simulink model "Copter_Plane_V10_sim"  (R2021a)
settings: Solver=ode1  StartTime=0.0  StopTime=10  FixedStep=dt  RelTol=1e-3
undefined symbols (not defined in the file or in its folder): AC_Attitude, AC_PosControl, accel_target, AP_Motors, curr_pos, Curr_sate, curr_vel, Euler, GRAVITY_MSS, gyro, HD, J, m_kg, Newton, pid_vel_xy_input, pos_target, position, Raphson, rho, SINS, SRV_Channel, Vehicle, vel_target, velocity
libraries: sharedutil x4, shared6dofsys x2, simulink x2, sharedtransform x2, aerolibasang x1
(part 1 of 2)
settings Model: PauseTimes=0.95  Creator=a4327481  LastModifiedBy=a4327481
settings SolverCC: AlgebraicLoopSolver=TrustRegion
settings DebuggingCC: SFMachineParentedDataDiag=warning

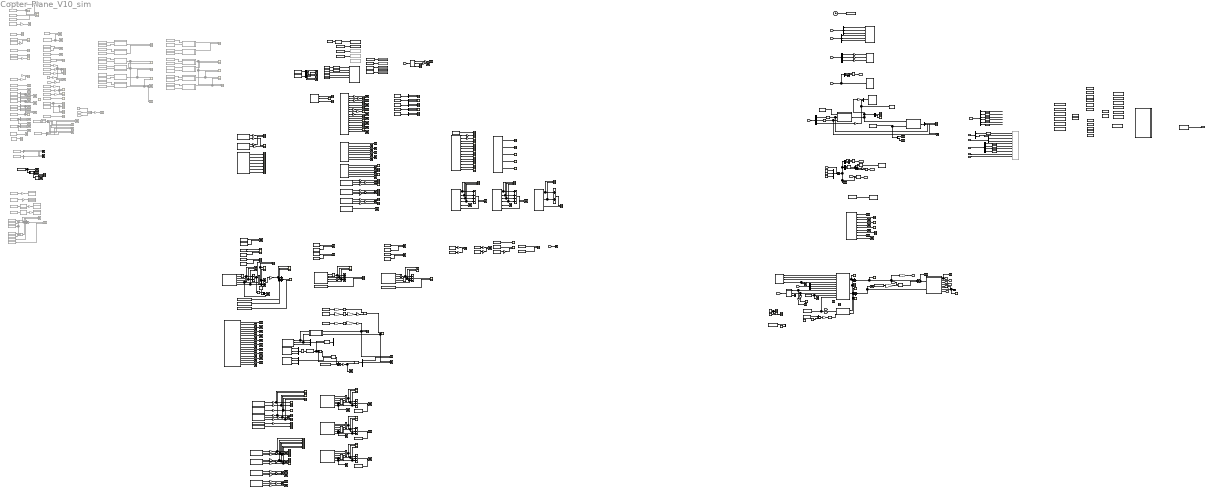
== system Copter_Plane_V10_sim ==
  CTRL_wp : Inport
  PathModeOut : Inport  Port=2  OutDataTypeStr=Bus: BUS_TASK_PATH_OutParam
  TASK_COMMON_OutParam : Inport  Port=3  OutDataTypeStr=Bus: BUS_TASK_COMMON_OutParam
  NAVI2CONTROL : Inport  Port=4  OutDataTypeStr=Bus: BUS_TO_CONTROL
  EAS_Algo : Inport  Port=5  OutDataTypeStr=Bus: BUS_AIRSPEED
  IMU : Inport  Port=6  OutDataTypeStr=Bus: BUS_IMU
  6DOF (Euler Angles) : Subsystem  AncestorBlock=shared6dof/6DOF (Euler Angles)  mask(6DOF EoM (Body Axis)){units=Metric (MKS), mtype=Fixed, rep=Euler Angles, xme_0=position, Vm_0=velocity, eul_0=Euler, pm_0=gyro, mass_0=m_kg, mass_e=0.5, mass_f=2.0, inertia=J, inertia_e=eye(3), inertia_f=2*eye(3), k_quat=1.0, vre_flag=on, abi_flag=off, aMode=0, xme_statename='', Vm_statename='', eul_statename='', quat_statename='', pm_statename='', mass_statename=''}
      mask prompts: units "shared_aeroblks:sharedaeroblk6dofbody:block6DOFEoMBodyAxisParamUnits"; mtype "shared_aeroblks:sharedaeroblk6dofbody:block6DOFEoMBodyAxisParamMasstype"; rep "shared_aeroblks:sharedaeroblk6dofbody:block6DOFEoMBodyAxisParamRepresentation"; xme_0 "shared_aeroblks:sharedaeroblk6dofbody:block6DOFEoMBodyAxisParamInitialpositionininertialaxesXeYeZe"; Vm_0 "shared_aeroblks:sharedaeroblk6dofbody:block6DOFEoMBodyAxisParamInitialvelocityinbodyaxesUvw"; eul_0 "shared_aeroblks:sharedaeroblk6dofbody:block6DOFEoMBodyAxisParamInitialEulerorientationrollpitchyaw"; pm_0 "shared_aeroblks:sharedaeroblk6dofbody:block6DOFEoMBodyAxisParamInitialbodyrotationratespqr"; mass_0 "shared_aeroblks:sharedaeroblk6dofbody:block6DOFEoMBodyAxisParamInitialmass"; mass_e "shared_aeroblks:sharedaeroblk6dofbody:block6DOFEoMBodyAxisParamEmptymass"; mass_f "shared_aeroblks:sharedaeroblk6dofbody:block6DOFEoMBodyAxisParamFullmass"; inertia "shared_aeroblks:sharedaeroblk6dofbody:block6DOFEoMBodyAxisParamInertia"; inertia_e "shared_aeroblks:sharedaeroblk6dofbody:block6DOFEoMBodyAxisParamEmptyinertiamatrix"; inertia_f "shared_aeroblks:sharedaeroblk6dofbody:block6DOFEoMBodyAxisParamFullinertiamatrix"; k_quat "shared_aeroblks:sharedaeroblk6dofbody:block6DOFEoMBodyAxisParamGainforquaternionnormalization"; vre_flag "shared_aeroblks:sharedaeroblk6dofbody:block6DOFEoMBodyAxisParamIncludemassflowrelativevelocity"; abi_flag "shared_aeroblks:sharedaeroblk6dofbody:inertialAccelFlag"; xme_statename "shared_aeroblks:sharedaeroblk6dofbody:block6DOFEoMStateNamePosition"; Vm_statename "shared_aeroblks:sharedaeroblk6dofbody:block6DOFEoMStateNameVelocity"; eul_statename "shared_aeroblks:sharedaeroblk6dofbody:block6DOFEoMStateNameEulerAngles"; quat_statename "shared_aeroblks:sharedaeroblk6dofbody:block6DOFEoMStateNameQuaternions"; pm_statename "shared_aeroblks:sharedaeroblk6dofbody:block6DOFEoMStateNameRotationRates"; mass_statename "shared_aeroblks:sharedaeroblk6dofbody:block6DOFEoMStateNameMass"
      mask help: shared_aeroblks:sharedaeroblk6dofbody:block6DOFEoMBodyAxisDesc
      mask init:
      | if aerosharedtest(gcb)
      |     ports=aerosharedicon('shared6dofbody','icon');
      | else
      |     ports=sharedautoicon('shared6dofbody','icon');
      | end
      mask Help: eval('aerosharedhelp(''sixdof_euler_angles'')');
      mask TypeOptions units: shared_aeroblks:sharedaeroblk6dofbody:block6DOFEoMBodyAxisParamComboMetricMKS | shared_aeroblks:sharedaeroblk6dofbody:block6DOFEoMBodyAxisParamComboEnglishVelocityinfts | shared_aeroblks:sharedaeroblk6dofbody:block6DOFEoMBodyAxisParamComboEnglishVelocityinkts
      mask TypeOptions mtype: shared_aeroblks:sharedaeroblk6dofbody:block6DOFEoMBodyAxisParamComboFixed | shared_aeroblks:sharedaeroblk6dofbody:block6DOFEoMBodyAxisParamComboSimpleVariable | shared_aeroblks:sharedaeroblk6dofbody:block6DOFEoMBodyAxisParamComboCustomVariable
      mask Callback mtype:
      | if aerosharedtest(gcb) && builtin('license','test','aerospace_blockset')
      |     aerosharedicon('shared6dofbody');
      | else
      |     sharedautoicon('shared6dofbody');
      | end
      mask TypeOptions rep: shared_aeroblks:sharedaeroblk6dofbody:block6DOFEoMBodyAxisParamComboEulerAngles | shared_aeroblks:sharedaeroblk6dofbody:block6DOFEoMBodyAxisParamComboQuaternion
      mask Callback rep:
      | if aerosharedtest(gcb) && builtin('license','test','aerospace_blockset')
      |     aerosharedicon('shared6dofbody');
      | else
      |     sharedautoicon('shared6dofbody');
      | end
      mask DialogControl Container4 Prompt: shared_aeroblks:sharedaeroblk6dofbody:block6DOFEoMParamTab
      mask DialogControl units Prompt: Units:
      mask DialogControl mtype Prompt: Mass type:
      mask DialogControl rep Prompt: Representation:
      mask DialogControl xme_0 Prompt: Initial position in inertial axes [Xe,Ye,Ze]:
      mask DialogControl Vm_0 Prompt: Initial velocity in body axes [U,v,w]:
      mask DialogControl eul_0 Prompt: Initial Euler orientation [roll, pitch, yaw]:
      mask DialogControl pm_0 Prompt: Initial body rotation rates [p,q,r]:
      mask DialogControl mass_0 Prompt: Initial mass:
      mask DialogControl mass_e Prompt: Empty mass:
      mask DialogControl mass_f Prompt: Full mass:
      mask DialogControl inertia Prompt: Inertia:
      mask DialogControl inertia_e Prompt: Empty inertia matrix:
      mask DialogControl inertia_f Prompt: Full inertia matrix:
      mask DialogControl k_quat Prompt: Gain for quaternion normalization:
      mask DialogControl vre_flag Prompt: Include mass flow relative velocity
      mask DialogControl abi_flag Prompt: Include inertial acceleration
      mask DialogControl Container6 Prompt: shared_aeroblks:sharedaeroblk6dofbody:block6DOFEoMStateAttributesTab
      mask DialogControl Container7 Prompt: shared_aeroblks:sharedaeroblk6dofbody:block6DOFEoMStateNamesGroup
      mask DialogControl xme_statename Prompt: Position: e.g., {'Xe', 'Ye', 'Ze'}
      mask DialogControl Vm_statename Prompt: Velocity: e.g., {'U', 'v', 'w'}
      mask DialogControl eul_statename Prompt: Euler rotation angles: e.g., {'phi', 'theta', 'psi'}
      mask DialogControl quat_statename Prompt: Quaternion vector: e.g., {'qr', 'qi', 'qj', 'qk'}
      mask DialogControl pm_statename Prompt: Body rotation rates: e.g., {'p', 'q', 'r'}
      mask DialogControl mass_statename Prompt: Mass: e.g., 'mass'
      mask Display:
      | port_label(ports(1).type,ports(1).port,ports(1).txt,'texmode','on');
      | port_label(ports(2).type,ports(2).port,ports(2).txt,'texmode','on');
      | port_label(ports(3).type,ports(3).port,ports(3).txt,'texmode','on');
      | port_label(ports(4).type,ports(4).port,ports(4).txt,'texmode','on');
      | port_label(ports(5).type,ports(5).port,ports(5).txt,'texmode','on');
      | port_label(ports(6).type,ports(6).port,ports(6).txt,'texmode','on');
      | port_label(ports(7).type,ports(7).port,ports(7).txt,'texmode','on');
      | port_label(ports(8).type,ports(8).port,ports(8).txt,'texmode','on');
      | port_label(ports(9).type,ports(9).port,ports(9).txt,'texmode','on');
      | port_label(ports(10).type,ports(10).port,ports(10).txt,'texmode','on');
      | port_label(ports(11).type,ports(11).port,ports(11).txt,'texmode','on');
      | port_label(ports(12).type,ports(12).port,ports(12).txt,'texmode','on');
      | port_label(ports(13).type,ports(13).port,ports(13).txt,'texmode','on');
      | port_label(ports(14).type,ports(14).port,ports(14).txt,'texmode','on');
      | port_label(ports(15).type,ports(15).port,ports(15).txt,'texmode','on');
      | port_label(ports(16).type,ports(16).port,ports(16).txt,'texmode','on');
      | port_label(ports(17).type,ports(17).port,ports(17).txt,'texmode','on');
  AC_Attitude : DataStoreMemory  DataStoreName=AC_Attitude  ReadBeforeWriteMsg=warning  WriteAfterWriteMsg=warning  WriteAfterReadMsg=warning  InitialValue=AC_Attitude  ShowAdditionalParam=off  OutDataTypeStr=Bus: BUS_CTRL_AC_Attitude
  AC_PosControl : DataStoreMemory  DataStoreName=AC_PosControl  ReadBeforeWriteMsg=warning  WriteAfterWriteMsg=warning  WriteAfterReadMsg=warning  InitialValue=AC_PosControl  ShowAdditionalParam=off  OutDataTypeStr=Bus: BUS_CTRL_AC_PosControl
  AC_rate_pitch_pid : DataStoreMemory  DataStoreName=AC_rate_pitch_pid  ReadBeforeWriteMsg=warning  WriteAfterWriteMsg=warning  WriteAfterReadMsg=warning  InitialValue=AC_rate_pitch_pid  ShowAdditionalParam=off  OutDataTypeStr=Bus: BUS_CTRL_PID
  AC_rate_roll_pid : DataStoreMemory  DataStoreName=AC_rate_roll_pid  ReadBeforeWriteMsg=warning  WriteAfterWriteMsg=warning  WriteAfterReadMsg=warning  InitialValue=AC_rate_roll_pid  ShowAdditionalParam=off  OutDataTypeStr=Bus: BUS_CTRL_PID
  AC_rate_yaw_pid : DataStoreMemory  DataStoreName=AC_rate_yaw_pid  ReadBeforeWriteMsg=warning  WriteAfterWriteMsg=warning  WriteAfterReadMsg=warning  InitialValue=AC_rate_yaw_pid  ShowAdditionalParam=off  OutDataTypeStr=Bus: BUS_CTRL_PID
  AP_L1 : DataStoreMemory  DataStoreName=AP_L1  ReadBeforeWriteMsg=warning  WriteAfterWriteMsg=warning  WriteAfterReadMsg=warning  InitialValue=AP_L1  ShowAdditionalParam=off  OutDataTypeStr=Bus: BUS_CTRL_AP_L1
  AP_Motors : DataStoreMemory  DataStoreName=AP_Motors  ReadBeforeWriteMsg=warning  WriteAfterWriteMsg=warning  WriteAfterReadMsg=warning  InitialValue=AP_Motors  VectorParams1D=off  ShowAdditionalParam=off  OutDataTypeStr=Bus: BUS_CTRL_AP_Motors
  AP_TECS : DataStoreMemory  DataStoreName=AP_TECS  ReadBeforeWriteMsg=warning  WriteAfterWriteMsg=warning  WriteAfterReadMsg=warning  InitialValue=AP_TECS  ShowAdditionalParam=off  OutDataTypeStr=Bus: BUS_CTRL_AP_TECS
  AP_rate_pitch : DataStoreMemory  DataStoreName=AP_rate_pitch  ReadBeforeWriteMsg=warning  WriteAfterWriteMsg=warning  WriteAfterReadMsg=warning  InitialValue=AP_rate_pitch  ShowAdditionalParam=off  OutDataTypeStr=Bus: BUS_CTRL_AP_PID_pitch
  AP_rate_roll : DataStoreMemory  DataStoreName=AP_rate_roll  ReadBeforeWriteMsg=warning  WriteAfterWriteMsg=warning  WriteAfterReadMsg=warning  InitialValue=AP_rate_roll  ShowAdditionalParam=off  OutDataTypeStr=Bus: BUS_CTRL_AP_PID_roll
  AP_rate_yaw : DataStoreMemory  DataStoreName=AP_rate_yaw  ReadBeforeWriteMsg=warning  WriteAfterWriteMsg=warning  WriteAfterReadMsg=warning  InitialValue=AP_rate_yaw  ShowAdditionalParam=off  OutDataTypeStr=Bus: BUS_CTRL_AP_PID_yaw
  Add : Sum  Inputs=++++
  Add{1,3,5,7,9,15..16} (7 alike) : Sum
  Add{4,6,10..13} (6 alike) : Sum  Inputs=+++
  Add14 : Sum  Inputs=++++
  Add2 : Sum  Commented=on  Inputs=+++
  Add8 : Sum  Inputs=+-
  Atan1 : Trigonometry  Operator=atan2
  Atan3 : Trigonometry  Operator=atan2
  Atan4 : Trigonometry  Operator=atan2
  Bus Selector : BusSelector  OutputSignals=curVelNED,curLLA
  Bus Selector1 : BusSelector  OutputSignals=pitchd,rolld,yawd,alt
  Bus Selector2 : BusSelector  OutputSignals=gyro_x,gyro_y,gyro_z,accel_x,accel_y,accel_z
  Bus Selector3 : BusSelector  OutputSignals=airspeed_indicate,EAS2TAS_Algo
  Clock : Clock
  Constant : Constant  Value=[40,100]*1e7
  Constant1 : Constant  Value=500/4500*0.95+0.05
  Constant10 : Constant  Value=500/4500*0.95+0.05
  Constant11 : Constant  Value=[40,100]*1e7
  Constant12 : Constant  Value=0
  Constant13 : Constant  Value=0
  Constant14 : Constant  Value=2  OutDataTypeStr=double
  Constant15 : Constant  Value=50  OutDataTypeStr=double
  Constant16 : Constant  OutDataTypeStr=double
  Constant17 : Constant  Value=[1750 1250 1750 1250]  VectorParams1D=off
  Constant2 : Constant  Value=1000  VectorParams1D=off
  Constant27 : Constant  Value=10  OutDataTypeStr=int16
  Constant3 : Constant  Value=[1 1 1 1]'
  Constant30 : Constant  Value=0
  Constant4 : Constant  Value=[1000 1000]
  Constant5 : Constant  Value=rho
  Constant6 : Constant  Value=4  OutDataTypeStr=int16
  Constant7 : Constant  Value=(1/rho)^0.5
  Constant8 : Constant  Value=11  OutDataTypeStr=int16
  Constant9 : Constant  Value=0.4
  Copter_Plane : DataStoreMemory  DataStoreName=Copter_Plane  ReadBeforeWriteMsg=warning  WriteAfterWriteMsg=warning  WriteAfterReadMsg=warning  InitialValue=Copter_Plane  VectorParams1D=off  ShowAdditionalParam=off  OutDataTypeStr=Bus: BUS_CTRL_Copter_Plane
  Curr_sate : DataStoreMemory  DataStoreName=Curr_sate  ReadBeforeWriteMsg=warning  WriteAfterWriteMsg=warning  WriteAfterReadMsg=warning  InitialValue=Curr_sate  VectorParams1D=off  ShowAdditionalParam=off  OutDataTypeStr=Bus: BUS_CTRL_Curr_sate
  Data Store Read : DataStoreRead  DataStoreName=SRV_Channel  IndexOptions=Index vector (dialog)  Indices=1  OutputSizes=1
  Data Store Read1 : DataStoreRead  DataStoreName=SINS  DataStoreElements=SINS.gyro_x#SINS.gyro_y#SINS.gyro_z#SINS.accel_x#SINS.accel_y#SINS.accel_z#SINS.roll#SINS.pitch#SINS.yaw#SINS.curr_vel(:,:)#SINS.curr_loc(:,:)#SINS.curr_alt#SINS.aspeed#SINS.EAS2TAS#SINS.groundspeed_vector(:,:)#SINS.curr_pos(:,:)#SINS.z_accel_meas  IndexOptions=Index vector (dialog)  Indices=1  OutputSizes=1
  Data Store Read10 : DataStoreRead  DataStoreName=AC_PosControl  DataStoreElements=AC_PosControl.vel_target(:,2)  IndexOptions=Index vector (dialog)  Indices=1  OutputSizes=1
  Data Store Read100 : DataStoreRead  DataStoreName=AP_rate_pitch  DataStoreElements=AP_rate_pitch.pid_info_P#AP_rate_pitch.pid_info_I#AP_rate_pitch.pid_info_D#AP_rate_pitch.pid_info_FF#AP_rate_pitch.pid_info_Dmod#AP_rate_pitch.last_out  IndexOptions=Index vector (dialog)  Indices=1  OutputSizes=1
  Data Store Read101 : DataStoreRead  DataStoreName=AP_rate_yaw  DataStoreElements=AP_rate_yaw.pid_info_I#AP_rate_yaw.pid_info_D#AP_rate_yaw.last_out  IndexOptions=Index vector (dialog)  Indices=1  OutputSizes=1
  Data Store Read102 : DataStoreRead  Commented=on  DataStoreName=pos_target  DataStoreElements=pos_target(:,1)  IndexOptions=Index vector (dialog)  Indices=1  OutputSizes=1
  Data Store Read103 : DataStoreRead  Commented=on  DataStoreName=curr_vel  DataStoreElements=curr_vel(:,1)  IndexOptions=Index vector (dialog)  Indices=1  OutputSizes=1
  Data Store Read104 : DataStoreRead  Commented=on  DataStoreName=curr_vel  DataStoreElements=curr_vel(:,2)  IndexOptions=Index vector (dialog)  Indices=1  OutputSizes=1
  Data Store Read105 : DataStoreRead  DataStoreName=AP_L1  DataStoreElements=AP_L1.L1_dist#AP_L1.last_Nu#AP_L1.latAccDem#AP_L1.nav_bearing#AP_L1.bearing_error  IndexOptions=Index vector (dialog)  Indices=1  OutputSizes=1
  Data Store Read106 : DataStoreRead  Commented=on  DataStoreName=thrust_error_angle  IndexOptions=Index vector (dialog)  Indices=1  OutputSizes=1
  Data Store Read107 : DataStoreRead  DataStoreName=AC_PosControl  DataStoreElements=AC_PosControl.accel_desired(:,:)  IndexOptions=Index vector (dialog)  Indices=1  OutputSizes=1
  Data Store Read108 : DataStoreRead  DataStoreName=AC_PosControl  DataStoreElements=AC_PosControl.accel_target(:,:)  IndexOptions=Index vector (dialog)  Indices=1  OutputSizes=1
  Data Store Read109 : DataStoreRead  DataStoreName=SINS  DataStoreElements=SINS.curr_vel(:,:)  IndexOptions=Index vector (dialog)  Indices=1  OutputSizes=1
  Data Store Read11 : DataStoreRead  DataStoreName=AC_PosControl  DataStoreElements=AC_PosControl.pos_target(:,2)  IndexOptions=Index vector (dialog)  Indices=1  OutputSizes=1
  Data Store Read110 : DataStoreRead  Commented=on  DataStoreName=nav_bearing  IndexOptions=Index vector (dialog)  Indices=1  OutputSizes=1
  Data Store Read111 : DataStoreRead  DataStoreName=SRV_Channel  DataStoreElements=SRV_Channel.k_rudder#SRV_Channel.k_aileron#SRV_Channel.k_throttle#SRV_Channel.k_elevator  IndexOptions=Index vector (dialog)  Indices=1  OutputSizes=1
  Data Store Read112 : DataStoreRead  DataStoreName=AC_PosControl  DataStoreElements=AC_PosControl.vel_target(:,:)  IndexOptions=Index vector (dialog)  Indices=1  OutputSizes=1
  Data Store Read113 : DataStoreRead  Commented=on  DataStoreName=mode_L1  IndexOptions=Index vector (dialog)  Indices=1  OutputSizes=1
  Data Store Read114 : DataStoreRead  DataStoreName=AC_PosControl  DataStoreElements=AC_PosControl.accel_target(:,3)  IndexOptions=Index vector (dialog)  Indices=1  OutputSizes=1
  Data Store Read115 : DataStoreRead  Commented=on  DataStoreName=pid_vel_xy_input  DataStoreElements=pid_vel_xy_input(:,1)  IndexOptions=Index vector (dialog)  Indices=1  OutputSizes=1
  Data Store Read116 : DataStoreRead  DataStoreName=SINS  DataStoreElements=SINS.z_accel_meas  IndexOptions=Index vector (dialog)  Indices=1  OutputSizes=1
  Data Store Read117 : DataStoreRead  DataStoreName=SINS  DataStoreElements=SINS.curr_vel(:,3)  IndexOptions=Index vector (dialog)  Indices=1  OutputSizes=1
  Data Store Read118 : DataStoreRead  DataStoreName=AC_PosControl  DataStoreElements=AC_PosControl.vel_desired(:,3)#AC_PosControl.vel_target(:,3)  IndexOptions=Index vector (dialog)  Indices=1  OutputSizes=1
  Data Store Read119 : DataStoreRead  DataStoreName=AC_PosControl  DataStoreElements=AC_PosControl.pos_target(:,3)  IndexOptions=Index vector (dialog)  Indices=1  OutputSizes=1
  Data Store Read12 : DataStoreRead  Commented=on  DataStoreName=pwm_out  IndexOptions=Index vector (dialog)  Indices=1  OutputSizes=1
  Data Store Read120 : DataStoreRead  DataStoreName=SINS  DataStoreElements=SINS.curr_alt  IndexOptions=Index vector (dialog)  Indices=1  OutputSizes=1
  Data Store Read121 : DataStoreRead  Commented=on  DataStoreName=z_accel_meas  IndexOptions=Index vector (dialog)  Indices=1  OutputSizes=1
  Data Store Read122 : DataStoreRead  Commented=on  DataStoreName=latAccDem  IndexOptions=Index vector (dialog)  Indices=1  OutputSizes=1
  Data Store Read123 : DataStoreRead  DataStoreName=AC_PosControl  DataStoreElements=AC_PosControl.vel_target(:,1)  IndexOptions=Index vector (dialog)  Indices=1  OutputSizes=1
  Data Store Read124 : DataStoreRead  DataStoreName=AC_PosControl  DataStoreElements=AC_PosControl.pos_target(:,1)  IndexOptions=Index vector (dialog)  Indices=1  OutputSizes=1
  Data Store Read125 : DataStoreRead  DataStoreName=SINS  DataStoreElements=SINS.curr_pos(:,1)  IndexOptions=Index vector (dialog)  Indices=1  OutputSizes=1
  Data Store Read126 : DataStoreRead  Commented=on  DataStoreName=pwm_out  IndexOptions=Index vector (dialog)  Indices=1  OutputSizes=1
  Data Store Read127 : DataStoreRead  Commented=on  DataStoreName=pos_target  IndexOptions=Index vector (dialog)  Indices=1  OutputSizes=1
  Data Store Read128 : DataStoreRead  Commented=on  DataStoreName=vel_target  IndexOptions=Index vector (dialog)  Indices=1  OutputSizes=1
  Data Store Read129 : DataStoreRead  Commented=on  DataStoreName=vel_desired  IndexOptions=Index vector (dialog)  Indices=1  OutputSizes=1
  Data Store Read13 : DataStoreRead  Commented=on  DataStoreName=thrust_rpyt_out  IndexOptions=Index vector (dialog)  Indices=1  OutputSizes=1
  Data Store Read130 : DataStoreRead  Commented=on  DataStoreName=accel_target  IndexOptions=Index vector (dialog)  Indices=1  OutputSizes=1
  Data Store Read131 : DataStoreRead  Commented=on  DataStoreName=accel_desired  IndexOptions=Index vector (dialog)  Indices=1  OutputSizes=1
  Data Store Read132 : DataStoreRead  DataStoreName=AP_Motors  DataStoreElements=AP_Motors.throttle_hover  IndexOptions=Index vector (dialog)  Indices=1  OutputSizes=1
  Data Store Read133 : DataStoreRead  Commented=on  DataStoreName=EAS_dem  IndexOptions=Index vector (dialog)  Indices=1  OutputSizes=1
  Data Store Read134 : DataStoreRead  Commented=on  DataStoreName=nav_pitch_cd  IndexOptions=Index vector (dialog)  Indices=1  OutputSizes=1
  Data Store Read135 : DataStoreRead  DataStoreName=AP_Motors  DataStoreElements=AP_Motors.throttle_in  IndexOptions=Index vector (dialog)  Indices=1  OutputSizes=1
  Data Store Read136 : DataStoreRead  Commented=on  DataStoreName=nav_roll_cd  IndexOptions=Index vector (dialog)  Indices=1  OutputSizes=1
  Data Store Read137 : DataStoreRead  DataStoreName=AP_Motors  DataStoreElements=AP_Motors.angle_boost  IndexOptions=Index vector (dialog)  Indices=1  OutputSizes=1
  Data Store Read138 : DataStoreRead  DataStoreName=AC_Attitude  DataStoreElements=AC_Attitude.rate_target_ang_vel(:,1)#AC_Attitude.rate_target_ang_vel(:,2)#AC_Attitude.rate_target_ang_vel(:,3)  IndexOptions=Index vector (dialog)  Indices=1  OutputSizes=1
  Data Store Read139 : DataStoreRead  DataStoreName=SINS  DataStoreElements=SINS.curr_pos(:,2)  IndexOptions=Index vector (dialog)  Indices=1  OutputSizes=1
  Data Store Read14 : DataStoreRead  DataStoreName=SRV_Channel  DataStoreElements=SRV_Channel.k_rudder#SRV_Channel.k_aileron#SRV_Channel.k_elevator#SRV_Channel.k_throttle#SRV_Channel.k_flap#SRV_Channel.tail_tilt#SRV_Channel.pwm_tail#SRV_Channel.pwm_out(:,:)  IndexOptions=Index vector (dialog)  Indices=1  OutputSizes=1
  Data Store Read140 : DataStoreRead  DataStoreName=SINS  DataStoreElements=SINS.curr_vel(:,2)  IndexOptions=Index vector (dialog)  Indices=1  OutputSizes=1
  Data Store Read141 : DataStoreRead  DataStoreName=SINS  DataStoreElements=SINS.gyro_x#SINS.gyro_y#SINS.gyro_z  IndexOptions=Index vector (dialog)  Indices=1  OutputSizes=1
  Data Store Read142 : DataStoreRead  DataStoreName=SINS  DataStoreElements=SINS.roll#SINS.pitch#SINS.yaw  IndexOptions=Index vector (dialog)  Indices=1  OutputSizes=1
  Data Store Read143 : DataStoreRead  Commented=on  DataStoreName=roll  IndexOptions=Index vector (dialog)  Indices=1  OutputSizes=1
  Data Store Read144 : DataStoreRead  DataStoreName=SINS  DataStoreElements=SINS.curr_alt  IndexOptions=Index vector (dialog)  Indices=1  OutputSizes=1
  Data Store Read145 : DataStoreRead  DataStoreName=SINS  DataStoreElements=SINS.aspeed  IndexOptions=Index vector (dialog)  Indices=1  OutputSizes=1
  Data Store Read146 : DataStoreRead  DataStoreName=AP_TECS  DataStoreElements=AP_TECS.TAS_dem_adj  IndexOptions=Index vector (dialog)  Indices=1  OutputSizes=1
  Data Store Read147 : DataStoreRead  DataStoreName=SRV_Channel  DataStoreElements=SRV_Channel.k_throttle  IndexOptions=Index vector (dialog)  Indices=1  OutputSizes=1
  Data Store Read148 : DataStoreRead  DataStoreName=AC_Attitude  DataStoreElements=AC_Attitude.attitude_target_ang_vel(:,1)#AC_Attitude.attitude_target_ang_vel(:,2)#AC_Attitude.attitude_target_ang_vel(:,3)  IndexOptions=Index vector (dialog)  Indices=1  OutputSizes=1
  Data Store Read149 : DataStoreRead  DataStoreName=AC_Attitude  DataStoreElements=AC_Attitude.attitude_target_quat(:,:)  IndexOptions=Index vector (dialog)  Indices=1  OutputSizes=1
  Data Store Read15 : DataStoreRead  DataStoreName=AP_Motors  DataStoreElements=AP_Motors.yaw_in  IndexOptions=Index vector (dialog)  Indices=1  OutputSizes=1
  Data Store Read150 : DataStoreRead  Commented=on  DataStoreName=pid_info_I_pitch  IndexOptions=Index vector (dialog)  Indices=1  OutputSizes=1
  Data Store Read151 : DataStoreRead  Commented=on  DataStoreName=last_out_pitch  IndexOptions=Index vector (dialog)  Indices=1  OutputSizes=1
  Data Store Read152 : DataStoreRead  DataStoreName=AC_Attitude  DataStoreElements=AC_Attitude.attitude_target_euler_rate(:,1)#AC_Attitude.attitude_target_euler_rate(:,2)#AC_Attitude.attitude_target_euler_rate(:,3)  IndexOptions=Index vector (dialog)  Indices=1  OutputSizes=1
  Data Store Read153 : DataStoreRead  Commented=on  DataStoreName=pid_vel_xy_input  DataStoreElements=pid_vel_xy_input(:,2)  IndexOptions=Index vector (dialog)  Indices=1  OutputSizes=1
  Data Store Read154 : DataStoreRead  DataStoreName=SlewLimiter  DataStoreElements=SlewLimiter.pos_event_stored#SlewLimiter.neg_event_stored#SlewLimiter.pos_event_index#SlewLimiter.neg_event_index#SlewLimiter.pos_event_ms(:,:)#SlewLimiter.neg_event_ms(:,:)#SlewLimiter.max_pos_slew_rate#SlewLimiter.max_neg_slew_rate#SlewLimiter.modifier_slew_rate#SlewLimiter.output_slew_rate#SlewLimiter.last_sample#SlewLimiter.slew_filter#SlewLimiter.N_EVENTS#SlewLimiter.max_pos_slew_event_ms#SlewLimiter.max_neg_slew_event_ms#SlewLimiter.MODIFIER_GAIN#SlewLimiter.WINDOW_MS#SlewLimiter.DERIVATIVE_CUTOFF_FREQ#SlewLimiter.slew_rate_max#SlewLimiter.slew_rate_tau  IndexOptions=Index vector (dialog)  Indices=1  OutputSizes=1
  Data Store Read158 : DataStoreRead  Commented=on  DataStoreName=attitude_target_quat  IndexOptions=Index vector (dialog)  Indices=1  OutputSizes=1
  Data Store Read159 : DataStoreRead  Commented=on  DataStoreName=rate_pitch_pid  DataStoreElements=rate_pitch_pid.kp  IndexOptions=Index vector (dialog)  Indices=1  OutputSizes=1
  Data Store Read16 : DataStoreRead  DataStoreName=SINS  DataStoreElements=SINS.aspeed  IndexOptions=Index vector (dialog)  Indices=1  OutputSizes=1
  Data Store Read160 : DataStoreRead  Commented=on  DataStoreName=rate_pitch_pid  DataStoreElements=rate_pitch_pid.error  IndexOptions=Index vector (dialog)  Indices=1  OutputSizes=1
  Data Store Read163 : DataStoreRead  Commented=on  DataStoreName=rate_pitch_pid  DataStoreElements=rate_pitch_pid.kd  IndexOptions=Index vector (dialog)  Indices=1  OutputSizes=1
  Data Store Read164 : DataStoreRead  Commented=on  DataStoreName=rate_pitch_pid  DataStoreElements=rate_pitch_pid.derivative  IndexOptions=Index vector (dialog)  Indices=1  OutputSizes=1
  Data Store Read165 : DataStoreRead  Commented=on  DataStoreName=rate_pitch_pid  DataStoreElements=rate_pitch_pid.integrator  IndexOptions=Index vector (dialog)  Indices=1  OutputSizes=1
  Data Store Read166 : DataStoreRead  DataStoreName=AC_PosControl  DataStoreElements=AC_PosControl.roll_target#AC_PosControl.pitch_target  IndexOptions=Index vector (dialog)  Indices=1  OutputSizes=1
  Data Store Read167 : DataStoreRead  DataStoreName=AC_Attitude  DataStoreElements=AC_Attitude.attitude_target_euler_angle(:,3)  IndexOptions=Index vector (dialog)  Indices=1  OutputSizes=1
  Data Store Read168 : DataStoreRead  Commented=on  DataStoreName=rate_pitch_pid  DataStoreElements=rate_pitch_pid.Dmod  IndexOptions=Index vector (dialog)  Indices=1  OutputSizes=1
  Data Store Read169 : DataStoreRead  Commented=on  DataStoreName=pitch_in  IndexOptions=Index vector (dialog)  Indices=1  OutputSizes=1
  Data Store Read17 : DataStoreRead  DataStoreName=SRV_Channel  DataStoreElements=SRV_Channel.pwm_out(:,1:2)  IndexOptions=Index vector (dialog)  Indices=1  OutputSizes=1
  Data Store Read171 : DataStoreRead  DataStoreName=SINS  DataStoreElements=SINS.accel_x#SINS.accel_y#SINS.accel_z  IndexOptions=Index vector (dialog)  Indices=1  OutputSizes=1
  Data Store Read172 : DataStoreRead  DataStoreName=AC_PosControl  DataStoreElements=AC_PosControl.accel_target(:,1)#AC_PosControl.accel_target(:,2)#AC_PosControl.accel_target(:,3)  IndexOptions=Index vector (dialog)  Indices=1  OutputSizes=1
  Data Store Read174 : DataStoreRead  DataStoreName=SINS  DataStoreElements=SINS.roll#SINS.pitch#SINS.yaw  IndexOptions=Index vector (dialog)  Indices=1  OutputSizes=1
  Data Store Read18 : DataStoreRead  DataStoreName=plane_mode  IndexOptions=Index vector (dialog)  Indices=1  OutputSizes=1
  Data Store Read19 : DataStoreRead  DataStoreName=AP_Motors  DataStoreElements=AP_Motors.thrust_rpyt_out(:,:)#AP_Motors.throttle_filter#AP_Motors.roll_in#AP_Motors.pitch_in#AP_Motors.yaw_in#AP_Motors.throttle_in  IndexOptions=Index vector (dialog)  Indices=1  OutputSizes=1
  Data Store Read2 : DataStoreRead  Commented=on  DataStoreName=pid_info_P_pitch  IndexOptions=Index vector (dialog)  Indices=1  OutputSizes=1
  Data Store Read20 : DataStoreRead  Commented=on  DataStoreName=pitch  IndexOptions=Index vector (dialog)  Indices=1  OutputSizes=1
  Data Store Read21 : DataStoreRead  DataStoreName=Test_w  DataStoreElements=Test_w.roll_in#Test_w.pitch_in#Test_w.yaw_in#Test_w.throttle_in#Test_w.k_rudder#Test_w.k_elevator#Test_w.k_throttle#Test_w.k_aileron#Test_w.k_flap#Test_w.out  IndexOptions=Index vector (dialog)  Indices=1  OutputSizes=1
  Data Store Read22 : DataStoreRead  DataStoreName=Plane  DataStoreElements=Plane.nav_roll_cd#Plane.nav_pitch_cd  IndexOptions=Index vector (dialog)  Indices=1  OutputSizes=1
  Data Store Read23 : DataStoreRead  DataStoreName=SINS  DataStoreElements=SINS.roll#SINS.pitch#SINS.yaw  IndexOptions=Index vector (dialog)  Indices=1  OutputSizes=1
  Data Store Read24 : DataStoreRead  DataStoreName=AP_rate_pitch  DataStoreElements=AP_rate_pitch.pid_info_target#AP_rate_pitch.pid_info_actual#AP_rate_pitch.pid_info_error#AP_rate_pitch.pid_info_P#AP_rate_pitch.pid_info_I#AP_rate_pitch.pid_info_FF#AP_rate_pitch.pid_info_D  IndexOptions=Index vector (dialog)  Indices=1  OutputSizes=1
  Data Store Read25 : DataStoreRead  DataStoreName=PathModeOut_sl  DataStoreElements=PathModeOut_sl.flightControlMode  IndexOptions=Index vector (dialog)  Indices=1  OutputSizes=1
  Data Store Read26 : DataStoreRead  DataStoreName=Copter_Plane  DataStoreElements=Copter_Plane.roll_target_pilot#Copter_Plane.pitch_target_pilot#Copter_Plane.climb_rate_cms  IndexOptions=Index vector (dialog)  Indices=1  OutputSizes=1
  Data Store Read27 : DataStoreRead  DataStoreName=AC_PosControl  DataStoreElements=AC_PosControl.accel_target(:,1)  IndexOptions=Index vector (dialog)  Indices=1  OutputSizes=1
  Data Store Read28 : DataStoreRead  DataStoreName=AC_PosControl  DataStoreElements=AC_PosControl.accel_target(:,2)  IndexOptions=Index vector (dialog)  Indices=1  OutputSizes=1
  Data Store Read29 : DataStoreRead  DataStoreName=AC_PosControl  DataStoreElements=AC_PosControl.pid_vel_xy.kp#AC_PosControl.pid_vel_xy.error(:,2)#AC_PosControl.pid_vel_xy.kd#AC_PosControl.pid_vel_xy.derivative(:,2)#AC_PosControl.pid_vel_xy.integrator(:,2)  IndexOptions=Index vector (dialog)  Indices=1  OutputSizes=1
  Data Store Read3 : DataStoreRead  DataStoreName=AC_rate_pitch_pid  DataStoreElements=AC_rate_pitch_pid.kp#AC_rate_pitch_pid.error#AC_rate_pitch_pid.kd#AC_rate_pitch_pid.derivative#AC_rate_pitch_pid.Dmod#AC_rate_pitch_pid.integrator  IndexOptions=Index vector (dialog)  Indices=1  OutputSizes=1
  Data Store Read30 : DataStoreRead  DataStoreName=AC_PosControl  DataStoreElements=AC_PosControl.pid_vel_xy.kp#AC_PosControl.pid_vel_xy.error(:,1)#AC_PosControl.pid_vel_xy.kd#AC_PosControl.pid_vel_xy.derivative(:,1)#AC_PosControl.pid_vel_xy.integrator(:,1)  IndexOptions=Index vector (dialog)  Indices=1  OutputSizes=1
  Data Store Read31 : DataStoreRead  DataStoreName=AC_Attitude  DataStoreElements=AC_Attitude.attitude_target_euler_angle(:,:)  IndexOptions=Index vector (dialog)  Indices=1  OutputSizes=1
  Data Store Read32 : DataStoreRead  DataStoreName=SRV_Channel  DataStoreElements=SRV_Channel.pwm_out(:,:)  IndexOptions=Index vector (dialog)  Indices=1  OutputSizes=1
  Data Store Read33 : DataStoreRead  Commented=on  DataStoreName=curr_vel  IndexOptions=Index vector (dialog)  Indices=1  OutputSizes=1
  Data Store Read34 : DataStoreRead  Commented=on  DataStoreName=hgt_rate_dem  IndexOptions=Index vector (dialog)  Indices=1  OutputSizes=1
  Data Store Read35 : DataStoreRead  Commented=on  DataStoreName=vel_target  IndexOptions=Index vector (dialog)  Indices=1  OutputSizes=1
  Data Store Read36 : DataStoreRead  Commented=on  DataStoreName=nav_roll_cd  IndexOptions=Index vector (dialog)  Indices=1  OutputSizes=1
  Data Store Read37 : DataStoreRead  Commented=on  DataStoreName=throttle_dem  IndexOptions=Index vector (dialog)  Indices=1  OutputSizes=1
  Data Store Read38 : DataStoreRead  Commented=on  DataStoreName=pitch_dem  IndexOptions=Index vector (dialog)  Indices=1  OutputSizes=1
  Data Store Read39 : DataStoreRead  Commented=on  DataStoreName=nav_pitch_cd  IndexOptions=Index vector (dialog)  Indices=1  OutputSizes=1
  Data Store Read4 : DataStoreRead  DataStoreName=AP_Motors  DataStoreElements=AP_Motors.pitch_in  IndexOptions=Index vector (dialog)  Indices=1  OutputSizes=1
  Data Store Read40 : DataStoreRead  Commented=on  DataStoreName=pitch  IndexOptions=Index vector (dialog)  Indices=1  OutputSizes=1
  Data Store Read41 : DataStoreRead  Commented=on  DataStoreName=pid_info_desired_pitch  IndexOptions=Index vector (dialog)  Indices=1  OutputSizes=1
  Data Store Read42 : DataStoreRead  Commented=on  DataStoreName=pid_info_actual_pitch  IndexOptions=Index vector (dialog)  Indices=1  OutputSizes=1
  Data Store Read43 : DataStoreRead  Commented=on  DataStoreName=hgt_dem_adj  IndexOptions=Index vector (dialog)  Indices=1  OutputSizes=1
  Data Store Read44 : DataStoreRead  Commented=on  DataStoreName=height  IndexOptions=Index vector (dialog)  Indices=1  OutputSizes=1
  Data Store Read45 : DataStoreRead  Commented=on  DataStoreName=hgt_dem_adj  IndexOptions=Index vector (dialog)  Indices=1  OutputSizes=1
  Data Store Read46 : DataStoreRead  Commented=on  DataStoreName=Vz  IndexOptions=Index vector (dialog)  Indices=1  OutputSizes=1
  Data Store Read47 : DataStoreRead  DataStoreName=AP_TECS  DataStoreElements=AP_TECS.hgt_dem_adj  IndexOptions=Index vector (dialog)  Indices=1  OutputSizes=1
  Data Store Read48 : DataStoreRead  Commented=on  DataStoreName=thrust_rpyt_out  IndexOptions=Index vector (dialog)  Indices=1  OutputSizes=1
  Data Store Read49 : DataStoreRead  DataStoreName=Plane  DataStoreElements=Plane.nav_roll_cd  IndexOptions=Index vector (dialog)  Indices=1  OutputSizes=1
  Data Store Read5 : DataStoreRead  DataStoreName=AC_rate_roll_pid  DataStoreElements=AC_rate_roll_pid.kp#AC_rate_roll_pid.error#AC_rate_roll_pid.kd#AC_rate_roll_pid.derivative#AC_rate_roll_pid.Dmod#AC_rate_roll_pid.integrator  IndexOptions=Index vector (dialog)  Indices=1  OutputSizes=1
  Data Store Read50 : DataStoreRead  Commented=on  DataStoreName=pitch_in  IndexOptions=Index vector (dialog)  Indices=1  OutputSizes=1
  Data Store Read51 : DataStoreRead  Commented=on  DataStoreName=pos_target  DataStoreElements=pos_target(:,2)  IndexOptions=Index vector (dialog)  Indices=1  OutputSizes=1
  Data Store Read52 : DataStoreRead  Commented=on  DataStoreName=vel_target  DataStoreElements=vel_target(:,1)  IndexOptions=Index vector (dialog)  Indices=1  OutputSizes=1
  Data Store Read53 : DataStoreRead  Commented=on  DataStoreName=pitch_target  IndexOptions=Index vector (dialog)  Indices=1  OutputSizes=1
  Data Store Read54 : DataStoreRead  Commented=on  DataStoreName=roll_target  IndexOptions=Index vector (dialog)  Indices=1  OutputSizes=1
  Data Store Read55 : DataStoreRead  Commented=on  DataStoreName=target_yaw_rate  IndexOptions=Index vector (dialog)  Indices=1  OutputSizes=1
  Data Store Read56 : DataStoreRead  DataStoreName=Copter_Plane  DataStoreElements=Copter_Plane.Mode  IndexOptions=Index vector (dialog)  Indices=1  OutputSizes=1
  Data Store Read57 : DataStoreRead  DataStoreName=AC_Attitude  DataStoreElements=AC_Attitude.attitude_target_euler_angle(:,1)#AC_Attitude.attitude_target_euler_angle(:,2)#AC_Attitude.attitude_target_euler_angle(:,3)  IndexOptions=Index vector (dialog)  Indices=1  OutputSizes=1
  Data Store Read58 : DataStoreRead  Commented=on  DataStoreName=tail_tilt  IndexOptions=Index vector (dialog)  Indices=1  OutputSizes=1
  Data Store Read59 : DataStoreRead  Commented=on  DataStoreName=accel_last_z_cms  IndexOptions=Index vector (dialog)  Indices=1  OutputSizes=1
  Data Store Read6 : DataStoreRead  DataStoreName=AP_Motors  DataStoreElements=AP_Motors.roll_in  IndexOptions=Index vector (dialog)  Indices=1  OutputSizes=1
  Data Store Read60 : DataStoreRead  DataStoreName=PathModeOut_sl  DataStoreElements=PathModeOut_sl.flightTaskMode  IndexOptions=Index vector (dialog)  Indices=1  OutputSizes=1
  Data Store Read61 : DataStoreRead  Commented=on  DataStoreName=vel_target  DataStoreElements=vel_target(:,2)  IndexOptions=Index vector (dialog)  Indices=1  OutputSizes=1
  Data Store Read62 : DataStoreRead  DataStoreName=AC_Attitude  DataStoreElements=AC_Attitude.attitude_target_euler_rate(:,1)#AC_Attitude.attitude_target_euler_rate(:,2)#AC_Attitude.attitude_target_euler_rate(:,3)  IndexOptions=Index vector (dialog)  Indices=1  OutputSizes=1
  Data Store Read63 : DataStoreRead  DataStoreName=AC_Attitude  DataStoreElements=AC_Attitude.attitude_target_ang_vel(:,1)#AC_Attitude.attitude_target_ang_vel(:,2)#AC_Attitude.attitude_target_ang_vel(:,3)  IndexOptions=Index vector (dialog)  Indices=1  OutputSizes=1
  Data Store Read64 : DataStoreRead  DataStoreName=AP_Motors  DataStoreElements=AP_Motors.thrust_rpyt_out(:,:)  IndexOptions=Index vector (dialog)  Indices=1  OutputSizes=1
  Data Store Read65 : DataStoreRead  DataStoreName=SINS  DataStoreElements=SINS.groundspeed_vector(:,:)  IndexOptions=Index vector (dialog)  Indices=1  OutputSizes=1
  Data Store Read66 : DataStoreRead  Commented=on  DataStoreName=yaw  IndexOptions=Index vector (dialog)  Indices=1  OutputSizes=1
  Data Store Read67 : DataStoreRead  Commented=on  DataStoreName=vel_forward_last_pct  IndexOptions=Index vector (dialog)  Indices=1  OutputSizes=1
  Data Store Read68 : DataStoreRead  DataStoreName=AC_PosControl  DataStoreElements=AC_PosControl.pos_target(:,:)  IndexOptions=Index vector (dialog)  Indices=1  OutputSizes=1
  Data Store Read69 : DataStoreRead  Commented=on  DataStoreName=tail_tilt  IndexOptions=Index vector (dialog)  Indices=1  OutputSizes=1
  Data Store Read7 : DataStoreRead  Commented=on  DataStoreName=pwm_tail  IndexOptions=Index vector (dialog)  Indices=1  OutputSizes=1
  Data Store Read70 : DataStoreRead  DataStoreName=Plane  DataStoreElements=Plane.nav_pitch_cd  IndexOptions=Index vector (dialog)  Indices=1  OutputSizes=1
  Data Store Read71 : DataStoreRead  DataStoreName=AC_PosControl  DataStoreElements=AC_PosControl.vel_desired(:,:)  IndexOptions=Index vector (dialog)  Indices=1  OutputSizes=1
  Data Store Read72 : DataStoreRead  Commented=on  DataStoreName=accel_target  DataStoreElements=accel_target(:,1)  IndexOptions=Index vector (dialog)  Indices=1  OutputSizes=1
  Data Store Read73 : DataStoreRead  Commented=on  DataStoreName=accel_target  DataStoreElements=accel_target(:,2)  IndexOptions=Index vector (dialog)  Indices=1  OutputSizes=1
  Data Store Read74 : DataStoreRead  DataStoreName=AC_PosControl  DataStoreElements=AC_PosControl.vel_target(:,:)  IndexOptions=Index vector (dialog)  Indices=1  OutputSizes=1
  Data Store Read75 : DataStoreRead  DataStoreName=SINS  DataStoreElements=SINS.roll  IndexOptions=Index vector (dialog)  Indices=1  OutputSizes=1
  Data Store Read76 : DataStoreRead  DataStoreName=AC_PosControl  DataStoreElements=AC_PosControl.pitch_target  IndexOptions=Index vector (dialog)  Indices=1  OutputSizes=1
  Data Store Read77 : DataStoreRead  Commented=on  DataStoreName=curr_pos  DataStoreElements=curr_pos(1)  IndexOptions=Index vector (dialog)  Indices=1  OutputSizes=1
  Data Store Read78 : DataStoreRead  Commented=on  DataStoreName=curr_pos  DataStoreElements=curr_pos(2)  IndexOptions=Index vector (dialog)  Indices=1  OutputSizes=1
  Data Store Read79 : DataStoreRead  Commented=on  DataStoreName=pid_info_D_pitch  IndexOptions=Index vector (dialog)  Indices=1  OutputSizes=1
  Data Store Read8 : DataStoreRead  DataStoreName=AC_PosControl  DataStoreElements=AC_PosControl.pid_accel_z.kp#AC_PosControl.pid_accel_z.error#AC_PosControl.pid_accel_z.kd#AC_PosControl.pid_accel_z.derivative#AC_PosControl.pid_accel_z.Dmod#AC_PosControl.pid_accel_z.integrator  IndexOptions=Index vector (dialog)  Indices=1  OutputSizes=1
  Data Store Read80 : DataStoreRead  Commented=on  DataStoreName=pid_vel_xy_input  DataStoreElements=pid_vel_xy_input(:,1)  IndexOptions=Index vector (dialog)  Indices=1  OutputSizes=1
  Data Store Read81 : DataStoreRead  Commented=on  DataStoreName=pid_vel_xy_input  DataStoreElements=pid_vel_xy_input(:,2)  IndexOptions=Index vector (dialog)  Indices=1  OutputSizes=1
  Data Store Read82 : DataStoreRead  DataStoreName=SINS  DataStoreElements=SINS.pitch  IndexOptions=Index vector (dialog)  Indices=1  OutputSizes=1
  Data Store Read83 : DataStoreRead  Commented=on  DataStoreName=gyro_y  IndexOptions=Index vector (dialog)  Indices=1  OutputSizes=1
  Data Store Read84 : DataStoreRead  Commented=on  DataStoreName=pos_target  DataStoreElements=pos_target(:,1)  IndexOptions=Index vector (dialog)  Indices=1  OutputSizes=1
  Data Store Read85 : DataStoreRead  Commented=on  DataStoreName=curr_vel  DataStoreElements=curr_vel(:,1)  IndexOptions=Index vector (dialog)  Indices=1  OutputSizes=1
  Data Store Read86 : DataStoreRead  Commented=on  DataStoreName=curr_vel  DataStoreElements=curr_vel(:,2)  IndexOptions=Index vector (dialog)  Indices=1  OutputSizes=1
  Data Store Read87 : DataStoreRead  Commented=on  DataStoreName=pos_target  DataStoreElements=pos_target(:,2)  IndexOptions=Index vector (dialog)  Indices=1  OutputSizes=1
  Data Store Read88 : DataStoreRead  Commented=on  DataStoreName=vel_target  DataStoreElements=vel_target(:,1)  IndexOptions=Index vector (dialog)  Indices=1  OutputSizes=1
  Data Store Read89 : DataStoreRead  Commented=on  DataStoreName=vel_target  DataStoreElements=vel_target(:,2)  IndexOptions=Index vector (dialog)  Indices=1  OutputSizes=1
  Data Store Read9 : DataStoreRead  DataStoreName=AC_rate_yaw_pid  DataStoreElements=AC_rate_yaw_pid.kp#AC_rate_yaw_pid.error#AC_rate_yaw_pid.kd#AC_rate_yaw_pid.derivative#AC_rate_yaw_pid.Dmod#AC_rate_yaw_pid.integrator  IndexOptions=Index vector (dialog)  Indices=1  OutputSizes=1
  Data Store Read90 : DataStoreRead  DataStoreName=SINS  DataStoreElements=SINS.curr_vel(:,1)  IndexOptions=Index vector (dialog)  Indices=1  OutputSizes=1
  Data Store Read91 : DataStoreRead  DataStoreName=AC_PosControl  DataStoreElements=AC_PosControl.roll_target  IndexOptions=Index vector (dialog)  Indices=1  OutputSizes=1
  Data Store Read92 : DataStoreRead  DataStoreName=AC_PosControl  DataStoreElements=AC_PosControl.pitch_target  IndexOptions=Index vector (dialog)  Indices=1  OutputSizes=1
  Data Store Read93 : DataStoreRead  Commented=on  DataStoreName=accel_target  DataStoreElements=accel_target(:,1)  IndexOptions=Index vector (dialog)  Indices=1  OutputSizes=1
  Data Store Read94 : DataStoreRead  Commented=on  DataStoreName=accel_target  DataStoreElements=accel_target(:,2)  IndexOptions=Index vector (dialog)  Indices=1  OutputSizes=1
  Data Store Read95 : DataStoreRead  Commented=on  DataStoreName=curr_pos  DataStoreElements=curr_pos(1)  IndexOptions=Index vector (dialog)  Indices=1  OutputSizes=1
  Data Store Read96 : DataStoreRead  Commented=on  DataStoreName=curr_pos  DataStoreElements=curr_pos(2)  IndexOptions=Index vector (dialog)  Indices=1  OutputSizes=1
  Data Store Read97 : DataStoreRead  DataStoreName=AP_TECS  DataStoreElements=AP_TECS.PITCHmaxf#AP_TECS.PITCHminf#AP_TECS.TAS_dem#AP_TECS.TAS_dem_adj#AP_TECS.TAS_rate_dem#AP_TECS.hgt_dem_adj#AP_TECS.hgt_rate_dem#AP_TECS.TAS_state#AP_TECS.climb_rate#AP_TECS.vel_dot#AP_TECS.throttle_dem#AP_TECS.integTHR_state#AP_TECS.ff_throttle#AP_TECS.pitch_dem  IndexOptions=Index vector (dialog)  Indices=1  OutputSizes=1
  Data Store Read98 : DataStoreRead  DataStoreName=Plane  DataStoreElements=Plane.scaling_speed  IndexOptions=Index vector (dialog)  Indices=1  OutputSizes=1
  Data Store Read99 : DataStoreRead  DataStoreName=AP_rate_roll  DataStoreElements=AP_rate_roll.pid_info_P#AP_rate_roll.pid_info_I#AP_rate_roll.pid_info_D#AP_rate_roll.pid_info_FF#AP_rate_roll.pid_info_Dmod#AP_rate_roll.last_out  IndexOptions=Index vector (dialog)  Indices=1  OutputSizes=1
  Data Store Write : DataStoreWrite  DataStoreName=Curr_sate  DataStoreElements=Curr_sate.PathModeOut.flightTaskMode#Curr_sate.PathModeOut.flightControlMode#Curr_sate.PathModeOut.heightCmd#Curr_sate.PathModeOut.maxClimbSpeed#Curr_sate.PathModeOut.rollCmd#Curr_sate.PathModeOut.headingCmd  IndexOptions=Index vector (dialog)  Indices=1  OutputSizes=1
  Data Store Write10 : DataStoreWrite  DataStoreName=Curr_sate  DataStoreElements=Curr_sate.NAV_alt  IndexOptions=Index vector (dialog)  Indices=1  OutputSizes=1
  Data Store Write11 : DataStoreWrite  DataStoreName=Curr_sate  DataStoreElements=Curr_sate.EAS2TAS_Algo  IndexOptions=Index vector (dialog)  Indices=1  OutputSizes=1
  Data Store Write12 : DataStoreWrite  DataStoreName=algo_remote_ct_st  DataStoreElements=algo_remote_ct_st.throttle  IndexOptions=Index vector (dialog)  Indices=1  OutputSizes=1
  Data Store Write13 : DataStoreWrite  DataStoreName=Curr_sate  DataStoreElements=Curr_sate.gyro_x#Curr_sate.gyro_y#Curr_sate.gyro_z#Curr_sate.accel_x#Curr_sate.accel_y#Curr_sate.accel_z  IndexOptions=Index vector (dialog)  Indices=1  OutputSizes=1
  Data Store Write14 : DataStoreWrite  Commented=on  DataStoreName=algo_remote_ct_st  DataStoreElements=algo_remote_ct_st.roll  IndexOptions=Index vector (dialog)  Indices=1  OutputSizes=1
  Data Store Write15 : DataStoreWrite  Commented=on  DataStoreName=algo_remote_ct_st  DataStoreElements=algo_remote_ct_st.tail_throttle_pwm  IndexOptions=Index vector (dialog)  Indices=1  OutputSizes=1
  Data Store Write2 : DataStoreWrite  Commented=on  DataStoreName=Curr_sate  DataStoreElements=Curr_sate.EAS_Algo#Curr_sate.EAS2TAS_Algo#Curr_sate.curVelNED(:,:)#Curr_sate.curLLA(:,:)#Curr_sate.pitchd#Curr_sate.rolld#Curr_sate.yawd#Curr_sate.NAV_alt#Curr_sate.PathModeOut#Curr_sate.wp_in(:,:)  IndexOptions=Index vector (dialog)  Indices=1  OutputSizes=1
  Data Store Write35 : DataStoreWrite  DataStoreName=algo_remote_ct_st  DataStoreElements=algo_remote_ct_st.Mode  IndexOptions=Index vector (dialog)  Indices=1  OutputSizes=1
  Data Store Write4 : DataStoreWrite  Commented=on  DataStoreName=algo_remote_ct_st  DataStoreElements=algo_remote_ct_st.pitch  IndexOptions=Index vector (dialog)  Indices=1  OutputSizes=1
  Data Store Write5 : DataStoreWrite  DataStoreName=systime  IndexOptions=Index vector (dialog)  Indices=1  OutputSizes=1
  Data Store Write6 : DataStoreWrite  DataStoreName=Curr_sate  DataStoreElements=Curr_sate.curLLA(:,:)  IndexOptions=Index vector (dialog)  Indices=1  OutputSizes=1
  Data Store Write7 : DataStoreWrite  DataStoreName=Curr_sate  DataStoreElements=Curr_sate.rolld#Curr_sate.pitchd#Curr_sate.yawd  IndexOptions=Index vector (dialog)  Indices=1  OutputSizes=1
  Data Store Write8 : DataStoreWrite  DataStoreName=Curr_sate  DataStoreElements=Curr_sate.curVelNED(:,:)  IndexOptions=Index vector (dialog)  Indices=1  OutputSizes=1
  Data Store Write9 : DataStoreWrite  DataStoreName=Curr_sate  DataStoreElements=Curr_sate.EAS_Algo  IndexOptions=Index vector (dialog)  Indices=1  OutputSizes=1
  Data Type Conversion{,1..11} (12 alike) : DataTypeConversion
  Data Type Conversion12 : DataTypeConversion  OutDataTypeStr=Enum: ENUM_FlightControlMode  RndMeth=Ceiling
  Data Type Conversion13 : DataTypeConversion  OutDataTypeStr=Enum: ENUM_FlightTaskMode  RndMeth=Ceiling
  Data Type Conversion14 : DataTypeConversion  OutDataTypeStr=Enum: ENUM_Mode  RndMeth=Ceiling
  Delay : Delay  DelayLength=1  InitialCondition=0
  Delay1 : Delay  DelayLength=1  InitialCondition=0
  Demux{1..2,14..15} (4 alike) : Demux  Commented=on
  Demux{3..4,9..10,12..13,17,20..22,24..25,37,41,44,46..47} (17 alike) : Demux  Outputs=3
  Demux{5..6,16,19,23,38,40} (7 alike) : Demux  Commented=on  Outputs=3
  Demux{36,42..43,45} (4 alike) : Demux  Outputs=2
  Derivative : Derivative
  Derivative1 : Derivative
  Derivative3 : Derivative
  Display{,2..4} (4 alike) : Display  Commented=on
  Display{1,5..7} (4 alike) : Display
  Divide{,4..5,12..16} (8 alike) : Product  Inputs=**
  Divide1 : Product  Inputs=/*
  Divide{6..11} (6 alike) : Product  Inputs=***
  Divide2 : Product  Commented=on  Inputs=***
  Divide3 : Product  Commented=on  Inputs=***
  From2 : From  Commented=on  GotoTag=theta
  From23 : From  Commented=on  GotoTag=yaw_gps
  From28 : From  Commented=on  GotoTag=yaw_w
  GRAVITY_MSS1 : DataStoreMemory  DataStoreName=GRAVITY_MSS  ReadBeforeWriteMsg=warning  WriteAfterWriteMsg=warning  WriteAfterReadMsg=warning  InitialValue=GRAVITY_MSS  VectorParams1D=off  ShowAdditionalParam=off  OutDataTypeStr=double
  Gain : Gain  Gain=1/1000
  Gain{1,3..5,14,29,38,40..41,52,56..57} (12 alike) : Gain  Commented=on  Gain=HD
  Gain{9..10,17,19,21} (5 alike) : Gain  Gain=0.01
  Gain{7..8,11..13,15..16,22,28,30..37,43..45,48..49,51,53..55,59..64,66..68,71..73,75,80..85} (45 alike) : Gain  Gain=HD
  Gain18 : Gain  Gain=1/100/HD
  Gain2 : Gain  Commented=on  Gain=1/100
  Gain20 : Gain  Gain=1/100/HD
  Gain23 : Gain  Gain=GRAVITY_MSS
  Gain24 : Gain  Gain=-100
  Gain25 : Gain  Gain=1/100/HD
  Gain26 : Gain  Commented=on  Gain=-1
  Gain27 : Gain  Gain=GRAVITY_MSS
  Gain{39,42,46..47} (4 alike) : Gain  Commented=on  Gain=0.01
  Gain50 : Gain  Gain=100
  Gain58 : Gain  Gain=-1
  Gain6 : Gain  Gain=-1
  Gain65 : Gain  Gain=0.001
  Gain69 : Gain  Gain=1e-7
  Gain70 : Gain  Gain=100
  Gain86 : Gain  Gain=1/100
  Gain87 : Gain  Gain=1/100
  Gravity in Earth Axes1 : Gain  Gain=1/m_kg  SaturateOnIntegerOverflow=on  OutDataTypeStr=Inherit: Same as input  ParamDataTypeStr=Inherit: Same as input
  Gravity in Earth Axes2 : Gain  Gain=m_kg  SaturateOnIntegerOverflow=on  OutDataTypeStr=Inherit: Same as input  ParamDataTypeStr=Inherit: Same as input
  HD1 : DataStoreMemory  DataStoreName=HD  ReadBeforeWriteMsg=warning  WriteAfterWriteMsg=warning  WriteAfterReadMsg=warning  InitialValue=HD  ShowAdditionalParam=off  OutDataTypeStr=double
  Hypot1 : Math  Operator=hypot  SaturateOnIntegerOverflow=on
  Hypot2 : Math  Operator=hypot  SaturateOnIntegerOverflow=on
  Hypot3 : Math  Operator=hypot  SaturateOnIntegerOverflow=on
  "Incidence, Sideslip & Airspeed2" : Subsystem  AncestorBlock=aerolibasang/Incidence, Sideslip, & Airspeed  mask(Incidence,Sideslip,&Airspeed){}
      mask help: aeroblks:aeroblkasang:blockIncidenceSideslipAirspeedDesc
      mask init:
      | aeroicon('aeroblk');
      mask Help: eval('asbhelp(''incidence_sideslip_and_airspeed'')');
      mask Display:
      | port_label('input',1,'V_b','texmode','on');
      | port_label('output',1,'\alpha','texmode','on');
      | port_label('output',2,'\beta','texmode','on');
      | port_label('output',3,'V','texmode','on');
  "Incidence, Sideslip & Airspeed3" : aerolibasang/Incidence, Sideslip, & Airspeed
  Inertial to Body4 : Product  Multiplication=Matrix(*)  InputSameDT=on  SaturateOnIntegerOverflow=on  OutDataTypeStr=Inherit: Same as first input
  Inertial to Body5 : Product  Multiplication=Matrix(*)  InputSameDT=on  SaturateOnIntegerOverflow=on  OutDataTypeStr=Inherit: Same as first input
  LOCATION_SCALING_FACTOR1 : DataStoreMemory  DataStoreName=LOCATION_SCALING_FACTOR  ReadBeforeWriteMsg=warning  WriteAfterWriteMsg=warning  WriteAfterReadMsg=warning  InitialValue=LOCATION_SCALING_FACTOR  VectorParams1D=off  ShowAdditionalParam=off  OutDataTypeStr=double
  LOCATION_SCALING_FACTOR_INV : DataStoreMemory  DataStoreName=LOCATION_SCALING_FACTOR_INV  ReadBeforeWriteMsg=warning  WriteAfterWriteMsg=warning  WriteAfterReadMsg=warning  InitialValue=LOCATION_SCALING_FACTOR_INV  VectorParams1D=off  ShowAdditionalParam=off  OutDataTypeStr=double
  Location_offset1 : MATLAB Function  TreatAsAtomicUnit=on
  MATLAB Function : MATLAB Function  Commented=on  TreatAsAtomicUnit=on
  MATLAB Function1 : MATLAB Function  TreatAsAtomicUnit=on
  MATLAB Function10 : MATLAB Function  Commented=on  TreatAsAtomicUnit=on
  MATLAB Function11 : MATLAB Function  Commented=on  TreatAsAtomicUnit=on
  MATLAB Function12 : MATLAB Function  Commented=on  TreatAsAtomicUnit=on
  MATLAB Function13 : MATLAB Function  Commented=on  TreatAsAtomicUnit=on
  MATLAB Function15 : MATLAB Function  Commented=on  TreatAsAtomicUnit=on
  MATLAB Function16 : MATLAB Function  Commented=on  TreatAsAtomicUnit=on
  MATLAB Function17 : MATLAB Function  TreatAsAtomicUnit=on
  MATLAB Function2 : MATLAB Function  Commented=on  TreatAsAtomicUnit=on
  MATLAB Function3 : MATLAB Function  Commented=on  TreatAsAtomicUnit=on
  MATLAB Function4 : MATLAB Function  Commented=on  TreatAsAtomicUnit=on
  MATLAB Function5 : MATLAB Function  Commented=on  TreatAsAtomicUnit=on
  MATLAB Function6 : MATLAB Function  Commented=on  TreatAsAtomicUnit=on
  MATLAB Function7 : MATLAB Function  Commented=on  TreatAsAtomicUnit=on
  MATLAB Function8 : MATLAB Function  Commented=on  TreatAsAtomicUnit=on
  MATLAB Function9 : MATLAB Function  Commented=on  TreatAsAtomicUnit=on
  Mux : Mux  Inputs=2
  Mux1 : Mux  Inputs=2
  Mux{3..4,7,10} (4 alike) : Mux  Inputs=3
  Mux2 : Mux  Inputs=2
  Mux5 : Mux  Commented=on  Inputs=3
  PathModeOut1 : DataStoreMemory  DataStoreName=PathModeOut_sl  ReadBeforeWriteMsg=warning  WriteAfterWriteMsg=warning  WriteAfterReadMsg=warning  InitialValue=PathModeOut_sl  VectorParams1D=off  ShowAdditionalParam=off  OutDataTypeStr=Bus: BUS_TASK_PATH_OutParam
  Plane : DataStoreMemory  DataStoreName=Plane  ReadBeforeWriteMsg=warning  WriteAfterWriteMsg=warning  WriteAfterReadMsg=warning  InitialValue=Plane  ShowAdditionalParam=off  OutDataTypeStr=Bus: BUS_CTRL_Plane
  Repeating Sequence : simulink/Sources/Repeating Sequence  rep_seq_t=[0 2]  rep_seq_y=[1050 2000]
  Rotation Angles to Direction Cosine Matrix1 : sharedtransform/Rotation Angles to Direction Cosine Matrix  rotationOrder=ZYX  aMode=aMode
      settings: SourceProductBaseCode=AE,PW,DR,MT,UV,VE
  SINS : DataStoreMemory  DataStoreName=SINS  ReadBeforeWriteMsg=warning  WriteAfterWriteMsg=warning  WriteAfterReadMsg=warning  InitialValue=SINS  VectorParams1D=off  ShowAdditionalParam=off  OutDataTypeStr=Bus: BUS_CTRL_SINS
  SRV_Channel : DataStoreMemory  DataStoreName=SRV_Channel  ReadBeforeWriteMsg=warning  WriteAfterWriteMsg=warning  WriteAfterReadMsg=warning  InitialValue=SRV_Channel  ShowAdditionalParam=off  OutDataTypeStr=Bus: BUS_CTRL_SRV_Channel
  Scope{,4,15..24,26..27,29..39,41..48,56,58..59,65..68,70..71,79,82,85..86,89..95,101,103..104,107..113,115..116,119..120,123,125,129..137,139,141,144,146,152,175,177..178,180..182,184..185,188..197,204..205,210..215,217..225,227,231..236,240..248,253..275} (157 alike) : Scope
  Scope{1,3,54,60,72,80..81,96..98,102,118,126..128,140,142,145,147,160,162} (21 alike) : Scope  Commented=on
  Scope{2,5,7,10,53,156,159,161,164..165,171,173,249} (13 alike) : Scope  NumInputPorts=3
  Scope{6,8..9,50..52,76..78,99..100,138,149,153,166..169,172,174,179,183,186..187,198..203,206..209,216,226,228..230,239,250..252} (43 alike) : Scope  NumInputPorts=2
  Scope{11..14,25,40,49,55,57,61..64,69,73..75,84,87..88,105,114,117,121..122,124,148,163,170,176} (30 alike) : Scope  Commented=on  NumInputPorts=2
  Scope{28,106,150..151,154,157..158} (7 alike) : Scope  Commented=on  NumInputPorts=3
  Scope143 : Scope  Commented=on  NumInputPorts=4
  Scope155 : Scope  Commented=on  NumInputPorts=4
  Scope237 : Scope  NumInputPorts=4
  Scope238 : Scope  NumInputPorts=4
  Scope83 : Scope  Commented=on  NumInputPorts=4
  Selector2 : Selector  InputPortWidth=3  IndexOptions=Index vector (dialog)  Indices=[3 2 1]  OutputSizes=1
  SlewLimiter : DataStoreMemory  DataStoreName=SlewLimiter  ReadBeforeWriteMsg=warning  WriteAfterWriteMsg=warning  WriteAfterReadMsg=warning  InitialValue=SlewLimiter  VectorParams1D=off  ShowAdditionalParam=off  OutDataTypeStr=Bus: BUS_CTRL_SlewLimiter
  Sqrt : Sqrt  SaturateOnIntegerOverflow=on
  Subsystem1 : Subsystem
  Sum1 : Sum
  Tan : Trigonometry  Operator=tan
  Tan1 : Trigonometry  Operator=tan
  Tan2 : Trigonometry  Operator=cos
  Terminator{1,8,10..11} (4 alike) : Terminator
  Test_w : DataStoreMemory  DataStoreName=Test_w  ReadBeforeWriteMsg=warning  WriteAfterWriteMsg=warning  WriteAfterReadMsg=warning  InitialValue=Test_w  ShowAdditionalParam=off  OutDataTypeStr=Bus: BUS_CTRL_Test_w
  Transpose3 : Math  Operator=transpose  SignedPower=on  SaturateOnIntegerOverflow=on
  algo_dbg_param : DataStoreMemory  DataStoreName=algo_dbg_param  ReadBeforeWriteMsg=warning  WriteAfterWriteMsg=warning  WriteAfterReadMsg=warning  InitialValue=algo_dbg_param  VectorParams1D=off  ShowAdditionalParam=off  OutDataTypeStr=Bus: BUS_CTRL_dbg_param
  algo_remote_ct_st : DataStoreMemory  DataStoreName=algo_remote_ct_st  ReadBeforeWriteMsg=warning  WriteAfterWriteMsg=warning  WriteAfterReadMsg=warning  InitialValue=algo_remote_ct_st  VectorParams1D=off  ShowAdditionalParam=off  OutDataTypeStr=Bus:BUS_CTRL_remote_ct_st
  attitude_error_vector : DataStoreRead  Commented=on  DataStoreName=attitude_error_vector  IndexOptions=Index vector (dialog)  Indices=1  OutputSizes=1
  b2e : Product  Multiplication=Matrix(*)  InputSameDT=on  SaturateOnIntegerOverflow=on  OutDataTypeStr=Inherit: Same as first input
  b2e2 : Product  Multiplication=Matrix(*)  InputSameDT=on  SaturateOnIntegerOverflow=on  OutDataTypeStr=Inherit: Same as first input
  dt1 : DataStoreMemory  DataStoreName=dt  ReadBeforeWriteMsg=warning  WriteAfterWriteMsg=warning  WriteAfterReadMsg=warning  InitialValue=dt  ShowAdditionalParam=off  OutDataTypeStr=double
  e2b : Product  Multiplication=Matrix(*)  InputSameDT=on  SaturateOnIntegerOverflow=on  OutDataTypeStr=Inherit: Same as first input
  get_vector_xy_from_origin_NE1 : MATLAB Function  TreatAsAtomicUnit=on
  gn2 : Constant  Value=[0;0;GRAVITY_MSS]
  gn3 : Constant  Value=[0;0;GRAVITY_MSS]
  input_euler_angle_roll_pitch_euler_rate_yaw : MATLAB Function  TreatAsAtomicUnit=on
  plane_mode : DataStoreMemory  DataStoreName=plane_mode  ReadBeforeWriteMsg=warning  WriteAfterWriteMsg=warning  WriteAfterReadMsg=warning  InitialValue=plane_mode  VectorParams1D=off  ShowAdditionalParam=off  OutDataTypeStr=Enum: ENUM_plane_mode
  rot_body_to_ned : DataStoreRead  Commented=on  DataStoreName=rot_body_to_ned  IndexOptions=Index vector (dialog)  Indices=1  OutputSizes=1
  systime : DataStoreMemory  DataStoreName=systime  ReadBeforeWriteMsg=warning  WriteAfterWriteMsg=warning  WriteAfterReadMsg=warning  InitialValue=systime  ShowAdditionalParam=off  OutDataTypeStr=double
  Out1 : Outport  OutDataTypeStr=Bus: BUS_CTRL_SRV_Channel
  wires:
  Data Store Read/1 -> Out1/1
  NAVI2CONTROL/1 -> Bus Selector1/1
  Bus Selector1/3 -> Data Type Conversion2/1  "<yawd>"
  Bus Selector/2 -> Data Store Write2/4  "<curLLA>"
  Bus Selector3/2 -> Data Type Conversion4/1  "<EAS2TAS_Algo>"
  Bus Selector2/2 -> Data Type Conversion6/1  "<gyro_y>"
  Bus Selector2/4 -> Data Type Conversion8/1  "<accel_x>"
  PathModeOut/1 -> Data Store Write2/9  "PathModeOut"
  Bus Selector2/6 -> Data Type Conversion10/1  "<accel_z>"
  Bus Selector2/1 -> Data Type Conversion5/1  "<gyro_x>"
  TASK_COMMON_OutParam/1 -> Bus Selector/1
  Bus Selector2/3 -> Data Type Conversion7/1  "<gyro_z>"
  CTRL_wp/1 -> Data Store Write2/10  "wp_in"
  Bus Selector/1 -> Data Store Write2/3  "<curVelNED>"
  EAS_Algo/1 -> Bus Selector3/1  "EAS_Algo"
  Bus Selector1/2 -> Data Type Conversion1/1  "<rolld>"
  Data Type Conversion4/1 -> Data Store Write2/2  "EAS2TAS_Algo"
  Data Type Conversion/1 -> Data Store Write2/5  "pitchd"
  Bus Selector1/4 -> Data Type Conversion11/1  "<alt>"
  Data Type Conversion2/1 -> Data Store Write2/7  "yawd"
  Data Type Conversion1/1 -> Data Store Write2/6  "rolld"
  Bus Selector1/1 -> Data Type Conversion/1  "<pitchd>"
  Data Type Conversion3/1 -> Data Store Write2/1  "EAS_Algo"
  Bus Selector3/1 -> Data Type Conversion3/1  "<airspeed_indicate>"
  Data Type Conversion5/1 -> ?  "gyro_x"
  Data Type Conversion6/1 -> ?  "gyro_y"
  IMU/1 -> Bus Selector2/1
  Data Type Conversion8/1 -> ?  "accel_x"
  Data Type Conversion11/1 -> Data Store Write2/8  "NAV_alt"
  Bus Selector2/5 -> Data Type Conversion9/1  "<accel_y>"
  Data Type Conversion7/1 -> ?  "gyro_z"
  Data Type Conversion9/1 -> ?  "accel_y"
  Data Type Conversion10/1 -> ?  "accel_z"
  Data Store Read96/1 -> MATLAB Function11/2(y_cmss)
  6DOF (Euler Angles)/1(Ve) -> Scope205/1, [Ve]
  Mux4/1 -> Sum1/2
  Data Store Read21/6 -> Scope35/1
  Data Store Read86/1 -> MATLAB Function7/2(y_cmss)
  MATLAB Function4/1(forward) -> Scope55/2, Scope62/1
  Divide/1 -> Scope41/1
  "Incidence, Sideslip & Airspeed3"/2 -> Gain37/1  "Beta"
  Data Store Read115/1 -> MATLAB Function10/1(x_cmss)
  Data Store Read89/1 -> MATLAB Function9/2(y_cmss)
  Data Store Read21/10 -> Scope39/1
  Data Store Read94/1 -> MATLAB Function13/2(y_cmss)
  MATLAB Function12/1(forward) -> Scope84/2
  Data Store Read104/1 -> MATLAB Function12/2(y_cmss)
  Sqrt/1 -> Subsystem1/4(Motor Commands)
  Subsystem1/1(Motor Forces) -> Add5/2, Scope48/1
  Data Store Read80/1 -> MATLAB Function4/1(x_cmss)
  Data Store Read61/1 -> MATLAB Function3/2(y_cmss)
  Data Store Read78/1 -> MATLAB Function5/2(y_cmss)
  Data Store Read73/1 -> MATLAB Function6/2(y_cmss)
  MATLAB Function6/1(forward) -> Scope57/2, Scope62/2
  "Incidence, Sideslip & Airspeed2"/2(Beta) -> MATLAB Function1/9(beta), Gain8/1  "Beta"
  Data Store Read84/1 -> MATLAB Function8/1(x_cmss)
  get_vector_xy_from_origin_NE1/1(vec_ne) -> Demux36/1
  Gain/1 -> Sqrt/1
  Demux47/2 -> Atan3/1
  Data Store Read21/8 -> Scope37/1
  Data Store Read21/4 -> Scope33/1
  Repeating Sequence/1 -> Divide/1, Scope29/1
  6DOF (Euler Angles)/7(pdot,qdot,rdot) -> Scope103/1, Terminator8/1
  Sum1/1 -> Demux46/1, Demux44/1, Scope139/1, Inertial to Body5/2  "Vwe"
  Data Store Read21/1 -> Scope30/1
  Data Store Read18/1 -> Display5/1
  Constant2/1 -> Add8/2
  Add8/1 -> Gain/1
  Data Store Read60/1 -> Display1/1
  MATLAB Function16/1(y) -> Gain57/1
  attitude_error_vector/1 -> Gain29/1
  Data Store Read158/1 -> MATLAB Function15/1(u)
  Data Store Read85/1 -> MATLAB Function7/1(x_cmss)
  MATLAB Function7/2(right) -> Scope75/2
  Data Store Read21/7 -> Scope36/1
  Data Store Read51/1 -> MATLAB Function2/2(y_cmss)
  "Incidence, Sideslip & Airspeed3"/3 -> Scope71/1
  Data Store Read103/1 -> MATLAB Function12/1(x_cmss)
  MATLAB Function13/2(right) -> Scope74/2, Scope64/1, Scope63/2
  Gain6/1 -> Atan1/1
  MATLAB Function3/1(forward) -> Scope84/1, Scope57/1, Scope55/1
  Data Store Read95/1 -> MATLAB Function11/1(x_cmss)
  Gain57/1 -> Display4/1
  Gain29/1 -> Display/1
  Data Store Read164/1 -> Divide3/2
  MATLAB Function9/2(right) -> Scope75/1, Scope63/1, Scope40/1
  [Xe] -> Demux41/1
  Data Store Read21/2 -> Scope31/1
  Divide2/1 -> Scope106/1, Add2/1  "P"
  Data Store Read165/1 -> Scope106/3, Add2/3  "I"
  Data Store Read169/1 -> Scope105/2
  Data Store Read52/1 -> MATLAB Function3/1(x_cmss)
  Add1/1 -> Scope204/1, 6DOF (Euler Angles)/1(Forces)
  Demux46/1 -> Atan4/2
  MATLAB Function8/2(right) -> Scope69/2
  Hypot2/1 -> Hypot1/2, Atan1/2
  Data Store Read16/1 -> Scope47/1, MATLAB Function1/10(V)
  Data Store Read93/1 -> MATLAB Function13/1(x_cmss)
  Data Store Read159/1 -> Divide2/1
  Data Store Read163/1 -> Divide3/1
  Data Store Read72/1 -> MATLAB Function6/1(x_cmss)
  Demux41/1 -> Delay/1
  Data Store Read87/1 -> MATLAB Function8/2(y_cmss)
  Gain56/1 -> Display3/1
  Demux20/1 -> MATLAB Function1/5(wx)
  Demux47/1 -> Atan3/2
  Data Store Read168/1 -> Divide2/3, Divide3/3
  Demux43/1 -> Scope110/1
  [DCM_be] -> Inertial to Body4/1
  Data Store Read21/9 -> Scope38/1
  Data Store Read21/3 -> Scope32/1
  Data Store Read88/1 -> MATLAB Function9/1(x_cmss)
  Constant3/1 -> Divide/2
  [Ve] -> Data Store Write8/1, Demux47/1
  Demux42/1 -> Scope58/1
  MATLAB Function2/1(forward) -> Scope61/1
  MATLAB Function1/2(M) -> Scope46/1, Add7/1
  Demux20/2 -> MATLAB Function1/6(wy)
  Data Store Read77/1 -> MATLAB Function5/1(x_cmss)
  Demux36/1 -> Scope99/1
  Demux20/3 -> MATLAB Function1/7(wz)
  MATLAB Function5/1(forward) -> Scope61/2
  [wb] -> Demux20/1
  MATLAB Function15/1(y) -> Gain56/1
  Demux43/2 -> Scope113/1
  "Incidence, Sideslip & Airspeed3"/1 -> Gain49/1  "alpha"
  6DOF (Euler Angles)/2(Xe) -> [Xe]
  Constant5/1 -> Subsystem1/2(Density), MATLAB Function1/11(rho)
  Gravity in Earth Axes2/1 -> Inertial to Body4/2
  Demux41/3 -> Gain58/1
  Location_offset1/1(current_loc) -> get_vector_xy_from_origin_NE1/1(loc), Gain69/1, Demux42/1
  Data Store Read102/1 -> MATLAB Function2/1(x_cmss)
  [Vb] -> "Incidence, Sideslip & Airspeed3"/1
  Demux47/3 -> Terminator11/1
  Demux44/2 -> Hypot2/2
  "Incidence, Sideslip & Airspeed2"/1(Alpha) -> MATLAB Function1/8(alpha), Gain7/1  "alpha"
  Demux46/3 -> Terminator10/1
  Data Store Read21/5 -> Scope34/1
  6DOF (Euler Angles)/8(Ab) -> [Abb]
  Gain52/1 -> Display2/1
  Data Store Read160/1 -> Divide2/2
  Atan1/1 -> [theta]
  Add7/1 -> Scope44/1, 6DOF (Euler Angles)/2(Moments)
  Constant12/1 -> Mux4/1
  ? -> Subsystem1/3(pqr), Scope43/1
  Data Store Read17/1 -> Mux/1
  MATLAB Function10/2(right) -> Scope40/2, Scope74/1
  [Vwb] -> "Incidence, Sideslip & Airspeed2"/1(Vb)
  Demux42/2 -> Scope85/1
  [DCM_be] -> Inertial to Body5/1
  Atan3/1 -> [yaw_gps]
  6DOF (Euler Angles)/4(DCM) -> [DCM_be]
  MATLAB Function1/1(F) -> Scope45/1, Add5/1
  [Ve] -> Sum1/1
  MATLAB Function11/2(right) -> Scope69/1
  Constant11/1 -> Demux43/1, get_vector_xy_from_origin_NE1/2(loc_origin)
  Demux36/2 -> Scope100/1
  gn3/1 -> Gravity in Earth Axes2/1
  6DOF (Euler Angles)/6(p,q,r) -> [wb]
  Demux44/1 -> Hypot2/1
  Inertial to Body5/1 -> [Vwb]
  Constant30/1 -> Mux4/3
  Clock/1 -> Data Store Write5/1
  Constant4/1 -> Mux/2
  6DOF (Euler Angles)/5(Vb) -> [Vb]
  Gain37/1 -> Scope68/1
  Gain49/1 -> Scope67/1
  Data Store Read111/1 -> MATLAB Function1/1(k_rudder)
  ? -> Subsystem1/1(Vb), Scope42/1
  Data Store Read106/1 -> Gain52/1
  Constant13/1 -> Mux4/2
  Demux46/2 -> Atan4/1
  Atan4/1 -> [yaw_w]
  Add2/1 -> Scope105/1
  6DOF (Euler Angles)/3(Euler) -> [euler]
  Data Store Read81/1 -> MATLAB Function4/2(y_cmss)
  Demux41/2 -> Delay1/1
  Divide3/1 -> Add2/2, Scope106/2  "D"
  Subsystem1/2(Motor Torques) -> Add7/2, Scope188/1
  Demux44/3 -> Hypot1/1, Gain6/1
  Data Store Read153/1 -> MATLAB Function10/2(y_cmss)
  rot_body_to_ned/1 -> MATLAB Function16/1(u)
  Inertial to Body4/1 -> Add1/2
  [wb] -> Demux17/1
  [euler] -> Demux37/1
  Demux17/3 -> Data Store Write13/3
  Demux17/2 -> Data Store Write13/2
  Demux17/1 -> Data Store Write13/1
  Demux10/1 -> Data Store Write13/4
  Demux10/2 -> Data Store Write13/5
  Demux10/3 -> Data Store Write13/6
  [accel] -> Demux10/1
  Demux37/1 -> Gain28/1
  Demux37/2 -> Gain44/1
  Demux37/3 -> Gain45/1
  Gain28/1 -> Data Store Write7/1
  Gain44/1 -> Data Store Write7/2
  Gain45/1 -> Data Store Write7/3
  Gain58/1 -> Mux1/2, Data Store Write10/1
  Constant7/1 -> Data Store Write11/1
  Data Store Read111/2 -> MATLAB Function1/2(k_aileron)
  Data Store Read111/3 -> MATLAB Function1/3(k_throttle)
  Data Store Read111/4 -> Scope56/1, MATLAB Function1/4(k_elevator)
  "Incidence, Sideslip & Airspeed2"/3(V) -> Terminator1/1
  Gravity in Earth Axes1/1 -> [accel]
  Add5/1 -> Scope/1, Gravity in Earth Axes1/1, Add1/1
  Data Store Read14/2 -> Scope107/1
  Data Store Read14/1 -> Scope120/1
  Data Store Read14/4 -> Scope109/1
  Data Store Read14/3 -> Scope108/1
  Data Store Read14/6 -> Scope133/1
  Data Store Read14/5 -> Scope125/1
  Data Store Read14/8 -> Scope15/1
  Data Store Read14/7 -> Scope136/1
  Data Store Read56/1 -> Display6/1
  Constant1/1 -> Data Store Write4/1
  Data Store Read57/1 -> Gain31/1
  Data Store Read57/2 -> Gain30/1
  Data Store Read57/3 -> Gain32/1
  Gain31/1 -> Scope22/1
  Gain30/1 -> Scope116/1
  Gain32/1 -> Scope119/1
  Gain35/1 -> Scope130/1
  Gain33/1 -> Scope129/1
  Gain34/1 -> Scope131/1
  Data Store Read62/3 -> Gain35/1
  Data Store Read62/2 -> Gain33/1
  Data Store Read62/1 -> Gain34/1
  Data Store Read63/1 -> Gain43/1
  Data Store Read63/2 -> Gain36/1
  Data Store Read63/3 -> Gain48/1
  Gain43/1 -> Scope146/1
  Gain36/1 -> Scope141/1
  Gain48/1 -> Scope144/1
  Data Store Read64/1 -> Scope152/1
  Constant9/1 -> Data Store Write12/1
  Data Store Read1/9 -> Gain61/1
  Data Store Read1/6 -> Scope92/1
  Data Store Read1/4 -> Scope178/1
  Data Store Read1/12 -> Scope17/1
  Data Store Read1/14 -> Scope23/1
  Data Store Read1/5 -> Scope86/1
  Data Store Read1/7 -> Gain59/1
  Data Store Read1/16 -> Scope27/1
  Data Store Read1/11 -> Scope24/1
  Data Store Read1/13 -> Scope19/1
  Data Store Read1/15 -> Scope26/1
  Data Store Read1/17 -> Scope66/1
  Data Store Read1/2 -> Gain63/1
  Data Store Read1/3 -> Gain64/1
  Data Store Read1/1 -> Gain62/1
  Gain64/1 -> Scope177/1
  Gain62/1 -> Scope65/1
  Gain63/1 -> Scope175/1
  Data Store Read1/8 -> Gain60/1
  Data Store Read1/10 -> Scope132/1
  Gain60/1 -> Scope115/1
  Gain59/1 -> Scope93/1
  Gain61/1 -> Scope123/1
  Constant10/1 -> Data Store Write14/1
  Data Store Read68/1 -> Demux3/1
  Data Store Read71/1 -> Demux4/1
  Data Store Read74/1 -> Demux9/1
  Data Store Read108/1 -> Demux12/1
  Data Store Read107/1 -> Demux13/1
  Demux3/1 -> Scope2/1
  Demux3/2 -> Scope2/2
  Demux3/3 -> Scope2/3
  Demux4/1 -> Scope159/1
  Demux4/2 -> Scope159/2
  Demux4/3 -> Scope159/3
  Demux9/1 -> Scope161/1
  Demux9/2 -> Scope161/2
  Demux9/3 -> Scope161/3
  Demux12/1 -> Scope164/1
  Demux12/2 -> Scope164/2
  Demux12/3 -> Scope164/3
  Demux13/1 -> Scope165/1
  Demux13/2 -> Scope165/2
  Demux13/3 -> Scope165/3
  Data Store Read114/1 -> Scope169/1
  Data Store Read116/1 -> Scope169/2
  Demux21/1 -> Scope167/1
  Demux22/3 -> Scope168/2
  Demux22/1 -> Scope167/2
  Demux22/2 -> Scope166/2
  Demux21/2 -> Scope166/1
  Data Store Read112/1 -> Demux21/1
  Data Store Read109/1 -> Demux22/1
  Demux21/3 -> Scope168/1
  Data Store Read117/1 -> Scope171/3
  Data Store Read118/1 -> Scope171/1
  Data Store Read119/1 -> Scope172/1
  Data Store Read120/1 -> Scope172/2
  Data Store Read13/1 -> Demux2/1
  Gain47/1 -> Scope117/2
  Data Store Read12/1 -> MATLAB Function/1(PWM)
  Demux38/1 -> Scope154/1
  Gain39/1 -> Scope73/1
  Demux15/4 -> Scope155/4
  Demux6/1 -> Scope50/1
  Data Store Read79/1 -> Scope83/2, Scope3/1  "D"
  Data Store Read122/1 -> Scope127/1
  Data Store Read41/1 -> Scope88/1
  Demux40/1 -> Scope158/1
  Data Store Read53/1 -> Gain46/1
  Data Store Read42/1 -> Scope88/2
  Hypot3/1 -> Derivative1/1, Scope138/1, Scope135/1
  Gain14/1 -> Scope140/1
  Gain4/1 -> Scope28/2
  Data Store Read110/1 -> Scope122/2, Scope60/1
  Demux14/1 -> Scope143/1
  Data Store Read44/1 -> Scope176/1
  Demux40/2 -> Scope158/2
  Data Store Read39/1 -> Gain42/1
  Demux19/3 -> Scope124/1, Scope151/3
  Data Store Read20/1 -> Gain4/1
  Gain3/1 -> Scope81/1
  Gain40/1 -> Scope72/1
  Demux1/1 -> Scope11/1
  Data Store Read129/1 -> Demux38/1
  Gain2/1 -> Scope163/2
  Data Store Read150/1 -> Scope83/3  "I"
  Data Store Read65/1 -> Demux45/1, Scope134/1
  Demux5/1 -> Scope50/2
  Data Store Read130/1 -> Demux23/1
  Gain38/1 -> Scope117/1, Scope73/2
  Gain41/1 -> Scope114/1, Scope87/2
  From2/1 -> Gain5/1
  Gain46/1 -> Scope114/2
  Data Store Read45/1 -> Scope176/2
  Demux23/1 -> Scope157/1
  Demux2/2 -> Scope12/2
  Demux19/2 -> Scope151/2
  Demux1/4 -> Scope14/1
  Data Store Read35/1 -> Demux6/1
  Data Store Read58/1 -> Scope126/1
  Data Store Read121/1 -> Scope121/2, Scope142/1
  Data Store Read151/1 -> Scope83/4
  Gain42/1 -> Scope28/1, Scope87/1
  Demux40/3 -> Scope158/3
  Data Store Read38/1 -> Gain40/1
  Data Store Read131/1 -> Demux40/1
  Demux38/3 -> Scope154/3
  Data Store Read46/1 -> Gain26/1
  Demux45/1 -> Hypot3/1
  Data Store Read83/1 -> Gain3/1
  Demux2/1 -> Scope11/2
  Demux45/2 -> Hypot3/2
  Data Store Read40/1 -> Gain41/1
  Demux16/1 -> Scope150/1
  Data Store Read113/1 -> Scope122/1, Scope102/1
  Mux5/1 -> Gain14/1
  Demux16/3 -> Scope25/1, Scope150/3
  Data Store Read7/1 -> Scope1/1
  Demux15/3 -> Scope155/3
  Data Store Read50/1 -> Scope98/1
  MATLAB Function/1(PWM_n) -> Demux1/1
  From23/1 -> Mux5/3
  Data Store Read54/1 -> Gain47/1
  Demux1/3 -> Scope13/1
  Data Store Read2/1 -> Scope83/1, Scope54/1  "P"
  Data Store Read133/1 -> Scope96/1
  Data Store Read127/1 -> Demux16/1
  Gain5/1 -> Scope28/3
  From28/1 -> Mux5/2
  Data Store Read134/1 -> Gain2/1
  Data Store Read66/1 -> Mux5/1
  Demux1/2 -> Scope12/1
  Demux15/2 -> Scope155/2
  Demux14/3 -> Scope143/3
  Data Store Read36/1 -> Gain39/1
  Demux14/2 -> Scope143/2
  Gain26/1 -> Scope170/2
  Demux6/2 -> Scope51/1
  Data Store Read59/1 -> Scope128/1
  Demux23/2 -> Scope157/2
  Demux19/1 -> Scope151/1
  Demux16/2 -> Scope150/2
  Data Store Read143/1 -> Gain38/1
  Demux15/1 -> Scope155/1
  Data Store Read55/1 -> Scope118/1
  Demux14/4 -> Scope143/4
  Demux2/3 -> Scope13/2
  Data Store Read136/1 -> Scope160/1
  Demux23/3 -> Scope121/1, Scope157/3
  Demux5/2 -> Scope51/2
  Data Store Read69/1 -> Scope148/1
  Data Store Read48/1 -> Scope97/1, Demux15/1
  Data Store Read34/1 -> Scope170/1
  Demux2/4 -> Scope14/2
  Gain1/1 -> Scope163/1
  Data Store Read37/1 -> Scope80/1
  Data Store Read128/1 -> Demux19/1
  Data Store Read126/1 -> Scope145/1, Demux14/1
  Derivative1/1 -> Scope138/2, Scope137/1
  ? -> Gain1/1
  Data Store Read33/1 -> Demux5/1
  Data Store Read43/1 -> Scope162/1
  Data Store Read67/1 -> Scope148/2, Scope147/1
  Demux38/2 -> Scope154/2
  Data Store Read135/1 -> Scope174/2
  Data Store Read8/1 -> Divide4/1
  Data Store Read8/2 -> Divide4/2
  Data Store Read8/3 -> Divide5/1
  Data Store Read8/4 -> Divide5/2
  Divide5/1 -> Scope173/2, Add9/2  "D"
  Divide4/1 -> Scope173/1, Add9/1  "P"
  Data Store Read132/1 -> Add10/2, Scope249/2
  Data Store Read137/1 -> Scope249/3, Add10/3
  Add10/1 -> Scope174/1
  Gain65/1 -> Scope249/1, Add10/1
  Data Store Read125/1 -> Scope179/2
  Data Store Read124/1 -> Scope179/1
  Data Store Read123/1 -> Scope78/1
  Data Store Read90/1 -> Scope78/2
  Delay/1 -> Location_offset1/2(ofs_north), Scope99/2
  Delay1/1 -> Scope100/2, Location_offset1/3(ofs_east)
  Constant/1 -> Location_offset1/1(center_WP)
  Data Store Read140/1 -> Scope183/2
  Data Store Read10/1 -> Scope183/1
  Data Store Read11/1 -> Scope8/1
  Data Store Read139/1 -> Scope8/2
  Mux1/1 -> Data Store Write6/1
  Add3/1 -> Gain70/1
  b2e/1 -> Add3/1
  Selector2/1 -> Rotation Angles to Direction Cosine Matrix1/1
  Transpose3/1 -> b2e/1
  gn2/1 -> Add3/2
  Mux7/1 -> Selector2/1
  Rotation Angles to Direction Cosine Matrix1/1 -> e2b/1, b2e2/1, Transpose3/1
  Data Store Read174/3 -> Mux7/3
  Data Store Read174/2 -> Mux7/2
  Data Store Read174/1 -> Mux7/1
  Data Store Read171/1 -> Mux3/1
  Data Store Read171/2 -> Mux3/2
  Data Store Read171/3 -> Mux3/3
  Mux3/1 -> b2e/2
  Demux24/1 -> Scope186/2
  Demux24/2 -> Scope187/2
  Gain70/1 -> b2e2/2, Scope184/1
  Data Store Read172/2 -> Mux10/2, MATLAB Function17/2(y_cmss)
  Data Store Read172/3 -> Mux10/3
  Mux10/1 -> e2b/2
  e2b/1 -> Demux25/1
  b2e2/1 -> Demux24/1
  Data Store Read76/1 -> Gain18/1
  Gain18/1 -> Tan/1
  Tan/1 -> Gain23/1
  Gain23/1 -> Gain24/1
  Gain24/1 -> Scope206/1
  Divide1/1 -> Scope207/1
  Gain50/1 -> Divide1/2
  Gain20/1 -> Tan2/1
  Tan2/1 -> Divide1/1
  Data Store Read92/1 -> Gain20/1
  Data Store Read91/1 -> Gain25/1
  Gain27/1 -> Gain50/1
  Gain25/1 -> Tan1/1
  Tan1/1 -> Gain27/1
  Data Store Read172/1 -> Mux10/1, MATLAB Function17/1(x_cmss)
  MATLAB Function17/1(forward) -> Scope186/1, Scope206/2
  MATLAB Function17/2(right) -> Scope187/1, Scope207/2
  Gain7/1 -> Scope59/1
  Gain8/1 -> Scope70/1
  Data Store Read22/1 -> Gain9/1
  Data Store Read23/1 -> Gain11/1
  Data Store Read22/2 -> Gain10/1
  Data Store Read23/2 -> Gain12/1
  Gain9/1 -> Scope76/1
  Gain10/1 -> Scope77/1
  Gain11/1 -> Scope76/2
  Gain12/1 -> Scope77/2
  Data Store Read24/1 -> Scope79/1
  Data Store Read24/2 -> Scope82/1
  Data Store Read24/3 -> Scope89/1
  Data Store Read24/4 -> Scope90/1
  Data Store Read24/5 -> Scope91/1
  Data Store Read24/6 -> Scope94/1
  Data Store Read24/7 -> Scope101/1
  Data Type Conversion12/1 -> Data Store Write/2
  Data Type Conversion13/1 -> Data Store Write/1
  Constant6/1 -> Data Type Conversion13/1
  Constant8/1 -> Data Type Conversion12/1
  Data Store Read25/1 -> Display7/1
  Data Store Read26/3 -> Scope21/1
  Data Store Read26/1 -> Scope4/1
  Data Store Read26/2 -> Scope20/1
  Data Store Read19/2 -> Scope16/1
  Data Store Read19/4 -> Scope95/1
  Data Store Read19/1 -> Scope111/1
  Data Store Read19/3 -> Scope18/1
  Data Store Read19/5 -> Scope112/1
  Data Store Read19/6 -> Scope104/1
  Data Store Read30/1 -> Divide12/1
  Data Store Read30/3 -> Divide13/1
  Divide12/1 -> Scope53/1, Add13/1  "P"
  Divide13/1 -> Add13/2, Scope53/2  "D"
  Data Store Read30/2 -> Divide12/2
  Add13/1 -> Scope149/1
  Data Store Read30/5 -> Scope53/3, Add13/3  "I"
  Data Store Read30/4 -> Divide13/2
  Data Store Read27/1 -> Scope149/2
  Data Store Read28/1 -> Scope153/2
  Data Store Read29/4 -> Divide15/2
  Data Store Read29/5 -> Add12/3, Scope156/3  "I"
  Add12/1 -> Scope153/1
  Data Store Read29/2 -> Divide14/2
  Divide15/1 -> Scope156/2, Add12/2  "D"
  Divide14/1 -> Add12/1, Scope156/1  "P"
  Data Store Read29/3 -> Divide15/1
  Data Store Read29/1 -> Divide14/1
  Gain69/1 -> Mux1/1
  Constant14/1 -> Data Store Write/4
  Constant15/1 -> Data Store Write/3
  Data Store Read118/2 -> Scope171/2
  Gain13/1 -> Scope185/1
  Gain86/1 -> Scope196/1, Scope198/1
  Data Store Read9/1 -> Divide10/1
  Gain82/1 -> Scope192/1, Scope199/2
  Data Store Read9/6 -> Scope10/3, Add11/3  "I"
  Data Store Read15/1 -> Scope52/2
  Divide8/1 -> Add6/1, Scope7/1  "P"
  Data Store Read6/1 -> Scope9/2
  Data Store Read3/3 -> Divide7/1
  Data Store Read31/1 -> Gain13/1
  Data Store Read9/2 -> Divide10/2
  Data Store Read5/1 -> Divide8/1
  Gain66/1 -> Scope202/1, Scope180/1
  Data Store Read3/6 -> Scope5/3, Add4/3  "I"
  Gain67/1 -> Scope201/1, Scope182/1
  Data Store Read4/1 -> Scope6/2
  Data Store Read142/1 -> Gain83/1
  Add11/1 -> Scope52/1
  Data Store Read5/6 -> Add6/3, Scope7/3  "I"
  Gain68/1 -> Scope203/1, Scope181/1
  Data Store Read9/5 -> Scope275/1, Divide10/3, Divide11/3
  Add4/1 -> Scope6/1
  Divide11/1 -> Scope10/2, Add11/2  "D"
  Data Store Read3/4 -> Divide7/2
  Data Store Read5/3 -> Divide9/1
  Divide9/1 -> Add6/2, Scope7/2  "D"
  Gain75/1 -> Scope189/1, Scope202/2
  Data Store Read5/5 -> Divide9/3, Divide8/3, Scope273/1
  Data Store Read5/2 -> Divide8/2
  Data Store Read5/4 -> Divide9/2
  Divide10/1 -> Scope10/1, Add11/1  "P"
  Divide7/1 -> Scope5/2, Add4/2  "D"
  Data Store Read9/4 -> Divide11/2
  Divide6/1 -> Scope5/1, Add4/1  "P"
  Data Store Read3/2 -> Divide6/2
  Data Store Read141/1 -> Gain80/1
  Data Store Read141/3 -> Gain81/1
  Data Store Read138/1 -> Gain67/1
  Gain87/1 -> Scope199/1, Scope197/1
  Data Store Read166/1 -> Gain86/1
  Data Store Read167/1 -> Gain85/1
  Data Store Read3/1 -> Divide6/1
  Gain85/1 -> Scope200/1, Scope195/1
  Data Store Read9/3 -> Divide11/1
  Gain83/1 -> Scope194/1, Scope198/2
  Gain81/1 -> Scope203/2, Scope190/1
  Data Store Read142/3 -> Gain84/1
  Data Store Read142/2 -> Gain82/1
  Gain84/1 -> Scope200/2, Scope193/1
  Data Store Read141/2 -> Gain75/1
  Data Store Read166/2 -> Gain87/1
  Add6/1 -> Scope9/1
  Gain80/1 -> Scope201/2, Scope191/1
  Data Store Read138/3 -> Gain68/1
  Data Store Read138/2 -> Gain66/1
  Data Store Read3/5 -> Scope274/1, Divide6/3, Divide7/3
  Hypot1/1 -> Data Store Write9/1
  Data Store Read75/1 -> Gain15/1
  Gain15/1 -> Scope208/2
  Data Store Read82/1 -> Gain16/1
  Gain16/1 -> Scope209/2
  Data Store Read70/1 -> Gain19/1
  Data Store Read49/1 -> Gain17/1
  Gain17/1 -> Scope208/1
  Gain19/1 -> Scope209/1
  Data Store Read97/1 -> Gain51/1
  Data Store Read97/2 -> Gain53/1
  Data Store Read97/3 -> Scope212/1
  Data Store Read97/4 -> Scope213/1
  Data Store Read97/5 -> Scope214/1
  Data Store Read97/6 -> Scope215/1
  Gain51/1 -> Scope210/1
  Gain53/1 -> Scope211/1
  Add/1 -> Scope216/1
  Data Store Read99/6 -> Scope216/2
  Data Store Read97/13 -> Scope223/1
  Data Store Read97/14 -> Scope224/1
  Data Store Read97/7 -> Scope217/1
  Data Store Read97/8 -> Scope218/1
  Data Store Read97/9 -> Scope219/1
  Data Store Read97/10 -> Scope220/1
  Data Store Read97/11 -> Scope221/1
  Data Store Read97/12 -> Scope222/1
  Data Store Read99/1 -> Scope237/1, Add/1  "P"
  Data Store Read99/2 -> Add/2, Scope237/2  "I"
  Data Store Read99/3 -> Scope237/3, Add/3  "D"
  Data Store Read99/4 -> Scope237/4, Add/4  "FF"
  Data Store Read99/5 -> Scope225/1
  Data Store Read100/5 -> Scope227/1
  Data Store Read100/4 -> Scope238/4, Add14/4  "FF"
  Data Store Read100/3 -> Scope238/3, Add14/3  "D"
  Data Store Read100/2 -> Scope238/2, Add14/2  "I"
  Data Store Read100/1 -> Scope238/1, Add14/1  "P"
  Data Store Read100/6 -> Scope226/2
  Add14/1 -> Scope226/1
  Data Store Read101/1 -> Scope229/1, Add15/1  "I"
  Data Store Read101/3 -> Scope228/2
  Data Store Read101/2 -> Scope229/2, Add15/2  "D"
  Data Store Read105/1 -> Scope231/1
  Data Store Read105/2 -> Scope232/1
  Data Store Read105/3 -> Scope233/1
  Data Store Read105/4 -> Scope234/1
  Data Store Read105/5 -> Scope235/1
  Data Store Read98/1 -> Scope236/1
  Add15/1 -> Scope228/1
  Data Store Read144/1 -> Gain21/1
  Gain21/1 -> Scope230/2
  Data Store Read47/1 -> Scope230/1
  Data Store Read146/1 -> Scope239/1
  Data Store Read145/1 -> Scope239/2
  Data Store Read147/1 -> Scope240/1
  [Xe] -> Scope241/1
  Constant16/1 -> Data Store Write/5
  Data Store Read148/2 -> Gain22/1
  Data Store Read148/3 -> Gain55/1
  Data Store Read148/1 -> Gain54/1
  Gain54/1 -> Scope244/1
  Gain22/1 -> Scope242/1
  Gain55/1 -> Scope243/1
  Data Store Read149/1 -> Scope245/1
  Gain73/1 -> Scope247/1
  Gain71/1 -> Scope246/1
  Gain72/1 -> Scope248/1
  Data Store Read152/1 -> Gain72/1
  Data Store Read152/3 -> Gain73/1
  Data Store Read152/2 -> Gain71/1
  Data Store Read32/1 -> Add8/1
  Data Store Read8/6 -> Scope173/3, Scope251/2, Add16/2  "I"
  Add9/1 -> Derivative/1, Scope252/1, Divide16/1
  Divide16/1 -> Derivative3/1, Add16/1, Scope252/2, Scope251/1  "PD"
  Add16/1 -> Gain65/1
  Data Store Read8/5 -> Scope250/2, Divide16/2
  Derivative/1 -> Mux2/1
  Derivative3/1 -> Mux2/2
  Mux2/1 -> Scope250/1
  Data Store Read154/1 -> Scope254/1
  Data Store Read154/2 -> Scope253/1
  Data Store Read154/3 -> Scope255/1
  Data Store Read154/5 -> Scope256/1
  Data Store Read154/4 -> Scope257/1
  Data Store Read154/6 -> Scope258/1
  Data Store Read154/8 -> Scope259/1
  Data Store Read154/10 -> Scope263/1
  Data Store Read154/12 -> Scope264/1
  Data Store Read154/14 -> Scope265/1
  Data Store Read154/16 -> Scope269/1
  Data Store Read154/18 -> Scope270/1
  Data Store Read154/20 -> Scope271/1
  Data Store Read154/7 -> Scope260/1
  Data Store Read154/9 -> Scope261/1
  Data Store Read154/11 -> Scope262/1
  Data Store Read154/13 -> Scope266/1
  Data Store Read154/15 -> Scope267/1
  Data Store Read154/17 -> Scope268/1
  Data Store Read154/19 -> Scope272/1
  Constant27/1 -> Data Type Conversion14/1
  Data Type Conversion14/1 -> Data Store Write35/1
